simulink model "Coil"  (R2021b)
settings: Solver=FixedStepAuto  StartTime=-6000e-6  StopTime=6000e-6  FixedStep=25e-6  RelTol=1e-3
libraries: simulink x1
(part 1 of 2)
settings Model: Creator=teja  LastModifiedBy=teja

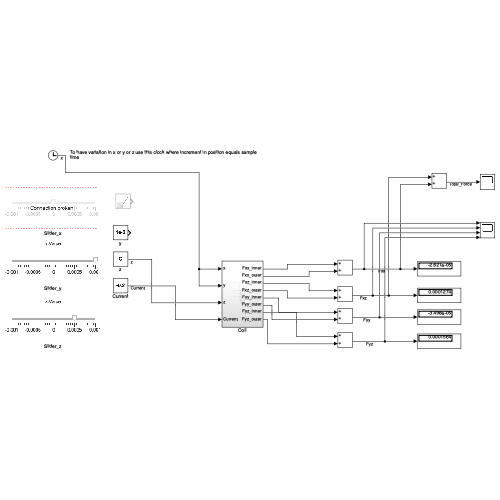
[thumbnail: Simulink's stored preview of the top-level diagram]
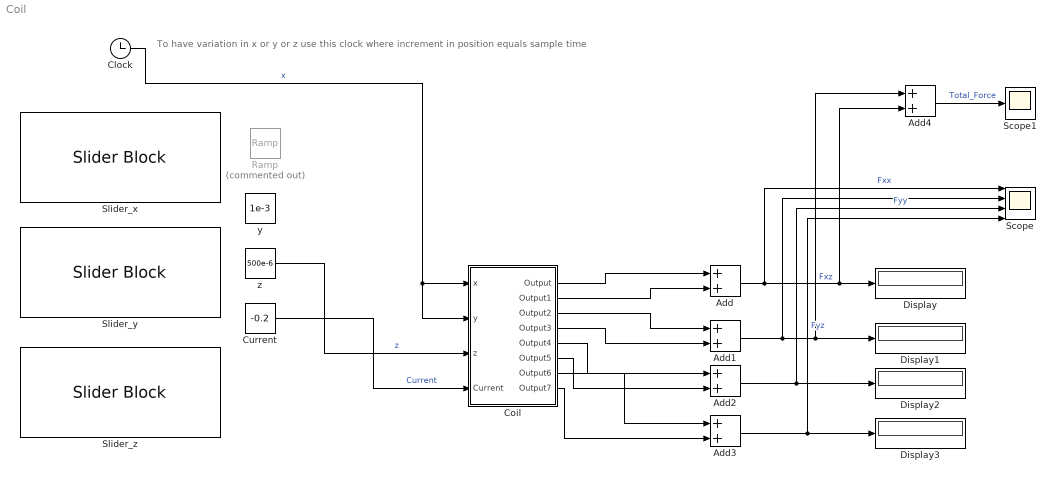
== system Coil ==
  note: To have variation in x or y or z use this clock where increment in position equals sample time
  Add{,1..4} (5 alike) : Sum
  Clock : Clock
  Coil : Subsystem
  Current : Constant  Value=-0.2
  Display{,1..3} (4 alike) : Display
  Ramp : simulink/Sources/Ramp  Commented=on  slope=1  start=0  InitialOutput=0
  Scope : Scope  NumInputPorts=4
  Scope1 : Scope
  Slider_x : SliderBlock  ScaleMin=-1000e-6  ScaleMax=1000e-6
  Slider_y : SliderBlock  ScaleMin=-1e-3  ScaleMax=1e-3
  Slider_z : SliderBlock  ScaleMin=-1000e-6  ScaleMax=1000e-6
  y : Constant  Value=1e-3
  z : Constant  Value=500e-6
  wires:
  Add/1 -> Add4/2, Display/1, Scope/1  "Fxx"
  Add1/1 -> Add4/1, Display1/1, Scope/2  "Fxz"
  Add2/1 -> Display2/1, Scope/3  "Fyy"
  Add3/1 -> Display3/1, Scope/4  "Fyz"
  Add4/1 -> Scope1/1  "Total_Force"
  z/1 -> Coil/3(z)  "z"
  Current/1 -> Coil/4(Current)  "Current"
  Coil/1(Output) -> Add/1
  Coil/2(Output1) -> Add/2
  Coil/3(Output2) -> Add1/1
  Coil/4(Output3) -> Add1/2
  Coil/5(Output4) -> Add2/1
  Coil/6(Output5) -> Add2/2
  Coil/7(Output6) -> Add3/1
  Coil/8(Output7) -> Add3/2
  Clock/1 -> Coil/1(x), Coil/2(y)  "x"

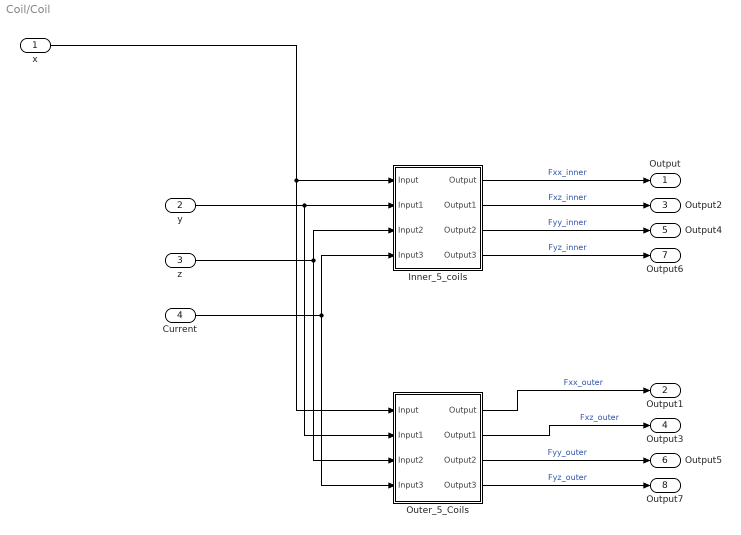
== system Coil/Coil ==
  x : Inport
  y : Inport  Port=2
  z : Inport  Port=3
  Current : Inport  Port=4
  Inner_5_coils : Subsystem
  Outer_5_Coils : Subsystem
  Output : Outport
  Output1 : Outport  Port=2
  Output2 : Outport  Port=3
  Output3 : Outport  Port=4
  Output4 : Outport  Port=5
  Output5 : Outport  Port=6
  Output6 : Outport  Port=7
  Output7 : Outport  Port=8
  wires:
  Outer_5_Coils/1(Output) -> Output1/1  "Fxx_outer"
  Inner_5_coils/4(Output3) -> Output6/1  "Fyz_inner"
  Outer_5_Coils/2(Output1) -> Output3/1  "Fxz_outer"
  y/1 -> Outer_5_Coils/2(Input1), Inner_5_coils/2(Input1)
  Outer_5_Coils/3(Output2) -> Output5/1  "Fyy_outer"
  z/1 -> Outer_5_Coils/3(Input2), Inner_5_coils/3(Input2)
  Inner_5_coils/2(Output1) -> Output2/1  "Fxz_inner"
  x/1 -> Outer_5_Coils/1(Input), Inner_5_coils/1(Input)
  Inner_5_coils/3(Output2) -> Output4/1  "Fyy_inner"
  Inner_5_coils/1(Output) -> Output/1  "Fxx_inner"
  Current/1 -> Outer_5_Coils/4(Input3), Inner_5_coils/4(Input3)
  Outer_5_Coils/4(Output3) -> Output7/1  "Fyz_outer"

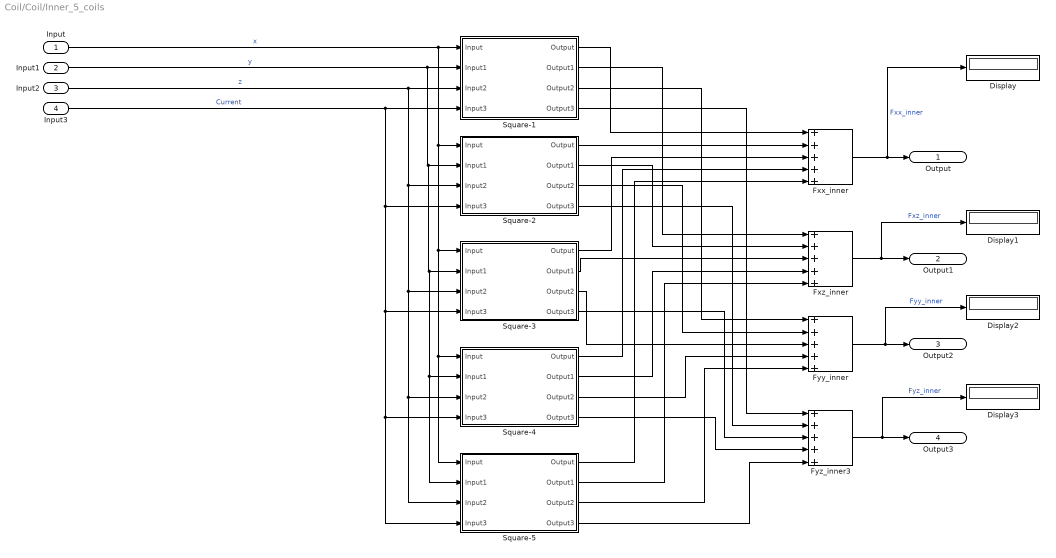
== system Coil/Coil/Inner_5_coils ==
  Input : Inport
  Input1 : Inport  Port=2
  Input2 : Inport  Port=3
  Input3 : Inport  Port=4
  Display{,1..3} (4 alike) : Display
  Fxx_inner : Sum  Inputs=+++++
  Fxz_inner : Sum  Inputs=+++++
  Fyy_inner : Sum  Inputs=+++++
  Fyz_inner3 : Sum  Inputs=+++++
  Square-1 : Subsystem
  Square-2 : Subsystem
  Square-3 : Subsystem
  Square-4 : Subsystem
  Square-5 : Subsystem
  Output : Outport
  Output1 : Outport  Port=2
  Output2 : Outport  Port=3
  Output3 : Outport  Port=4
  wires:
  Input/1 -> Square-5/1(Input), Square-4/1(Input), Square-3/1(Input), Square-2/1(Input), Square-1/1(Input)  "x"
  Input3/1 -> Square-2/4(Input3), Square-3/4(Input3), Square-4/4(Input3), Square-5/4(Input3), Square-1/4(Input3)  "Current"
  Input1/1 -> Square-5/2(Input1), Square-4/2(Input1), Square-3/2(Input1), Square-2/2(Input1), Square-1/2(Input1)  "y"
  Input2/1 -> Square-1/3(Input2), Square-3/3(Input2), Square-4/3(Input2), Square-5/3(Input2), Square-2/3(Input2)  "z"
  Square-1/1(Output) -> Fxx_inner/1
  Square-2/1(Output) -> Fxx_inner/2
  Square-3/1(Output) -> Fxx_inner/3
  Square-4/1(Output) -> Fxx_inner/4
  Square-5/1(Output) -> Fxx_inner/5
  Fxx_inner/1 -> Display/1, Output/1  "Fxx_inner"
  Fxz_inner/1 -> Display1/1, Output1/1  "Fxz_inner"
  Fyy_inner/1 -> Display2/1, Output2/1  "Fyy_inner"
  Fyz_inner3/1 -> Display3/1, Output3/1  "Fyz_inner"
  Square-1/2(Output1) -> Fxz_inner/1
  Square-2/2(Output1) -> Fxz_inner/2
  Square-3/2(Output1) -> Fxz_inner/3
  Square-4/2(Output1) -> Fxz_inner/4
  Square-5/2(Output1) -> Fxz_inner/5
  Square-1/3(Output2) -> Fyy_inner/1
  Square-2/3(Output2) -> Fyy_inner/2
  Square-3/3(Output2) -> Fyy_inner/3
  Square-4/3(Output2) -> Fyy_inner/4
  Square-5/3(Output2) -> Fyy_inner/5
  Square-1/4(Output3) -> Fyz_inner3/1
  Square-2/4(Output3) -> Fyz_inner3/2
  Square-3/4(Output3) -> Fyz_inner3/3
  Square-4/4(Output3) -> Fyz_inner3/4
  Square-5/4(Output3) -> Fyz_inner3/5

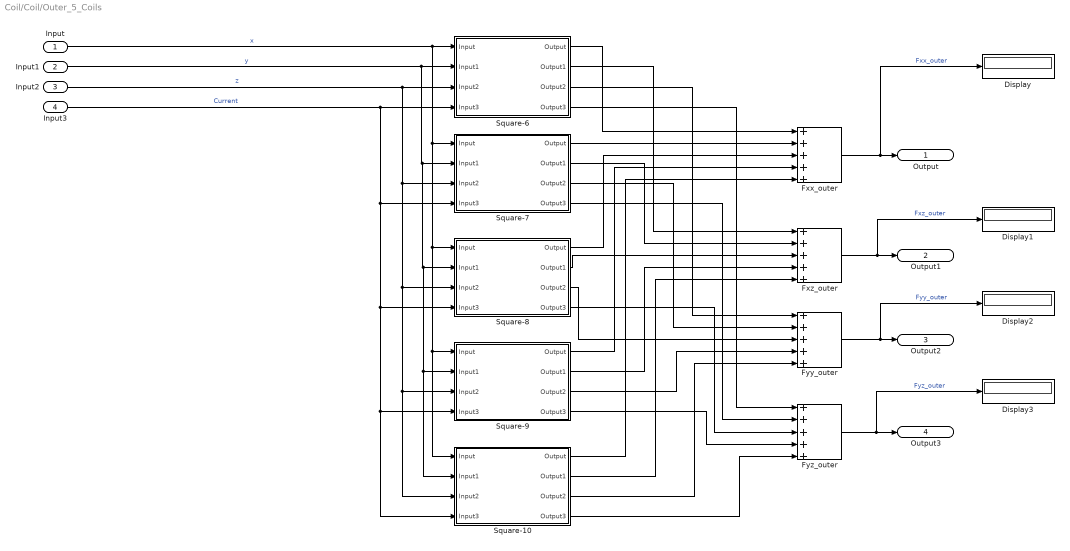
== system Coil/Coil/Outer_5_Coils ==
  Input : Inport
  Input1 : Inport  Port=2
  Input2 : Inport  Port=3
  Input3 : Inport  Port=4
  Display{,1..3} (4 alike) : Display
  Fxx_outer : Sum  Inputs=+++++
  Fxz_outer : Sum  Inputs=+++++
  Fyy_outer : Sum  Inputs=+++++
  Fyz_outer : Sum  Inputs=+++++
  Square-10 : Subsystem
  Square-6 : Subsystem
  Square-7 : Subsystem
  Square-8 : Subsystem
  Square-9 : Subsystem
  Output : Outport
  Output1 : Outport  Port=2
  Output2 : Outport  Port=3
  Output3 : Outport  Port=4
  wires:
  Square-10/4(Output3) -> Fyz_outer/5
  Square-9/4(Output3) -> Fyz_outer/4
  Square-8/4(Output3) -> Fyz_outer/3
  Square-7/4(Output3) -> Fyz_outer/2
  Square-6/4(Output3) -> Fyz_outer/1
  Square-10/3(Output2) -> Fyy_outer/5
  Square-9/3(Output2) -> Fyy_outer/4
  Square-8/3(Output2) -> Fyy_outer/3
  Square-7/3(Output2) -> Fyy_outer/2
  Square-6/3(Output2) -> Fyy_outer/1
  Square-10/2(Output1) -> Fxz_outer/5
  Square-9/2(Output1) -> Fxz_outer/4
  Square-8/2(Output1) -> Fxz_outer/3
  Square-7/2(Output1) -> Fxz_outer/2
  Square-6/2(Output1) -> Fxz_outer/1
  Fyz_outer/1 -> Display3/1, Output3/1  "Fyz_outer"
  Fyy_outer/1 -> Display2/1, Output2/1  "Fyy_outer"
  Fxz_outer/1 -> Display1/1, Output1/1  "Fxz_outer"
  Fxx_outer/1 -> Display/1, Output/1  "Fxx_outer"
  Square-10/1(Output) -> Fxx_outer/5
  Square-9/1(Output) -> Fxx_outer/4
  Square-8/1(Output) -> Fxx_outer/3
  Square-7/1(Output) -> Fxx_outer/2
  Square-6/1(Output) -> Fxx_outer/1
  Input2/1 -> Square-7/3(Input2), Square-10/3(Input2), Square-9/3(Input2), Square-8/3(Input2), Square-6/3(Input2)  "z"
  Input1/1 -> Square-6/2(Input1), Square-7/2(Input1), Square-8/2(Input1), Square-9/2(Input1), Square-10/2(Input1)  "y"
  Input3/1 -> Square-6/4(Input3), Square-10/4(Input3), Square-9/4(Input3), Square-8/4(Input3), Square-7/4(Input3)  "Current"
  Input/1 -> Square-6/1(Input), Square-7/1(Input), Square-8/1(Input), Square-9/1(Input), Square-10/1(Input)  "x"

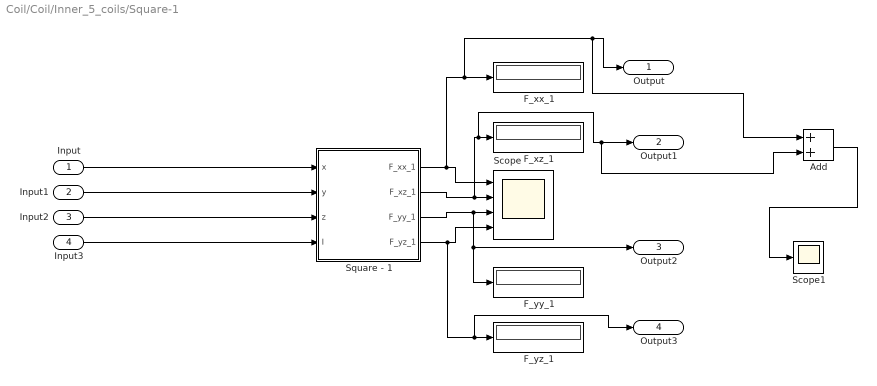
== system Coil/Coil/Inner_5_coils/Square-1 ==
  Input : Inport
  Input1 : Inport  Port=2
  Input2 : Inport  Port=3
  Input3 : Inport  Port=4
  Add : Sum
  F_xx_1 : Display
  F_xz_1 : Display
  F_yy_1 : Display
  F_yz_1 : Display
  Scope : Scope  NumInputPorts=4
  Scope1 : Scope
  Square - 1 : MATLAB Function  TreatAsAtomicUnit=on
  Output : Outport
  Output1 : Outport  Port=2
  Output2 : Outport  Port=3
  Output3 : Outport  Port=4
  wires:
  Square - 1/2(F_xz_1) -> Add/2, Output1/1, F_xz_1/1, Scope/2
  Square - 1/3(F_yy_1) -> F_yy_1/1, Output2/1, Scope/3
  Square - 1/1(F_xx_1) -> Add/1, Output/1, F_xx_1/1, Scope/1
  Square - 1/4(F_yz_1) -> Scope/4, Output3/1, F_yz_1/1
  Input/1 -> Square - 1/1(x)
  Input1/1 -> Square - 1/2(y)
  Input2/1 -> Square - 1/3(z)
  Input3/1 -> Square - 1/4(I)
  Add/1 -> Scope1/1

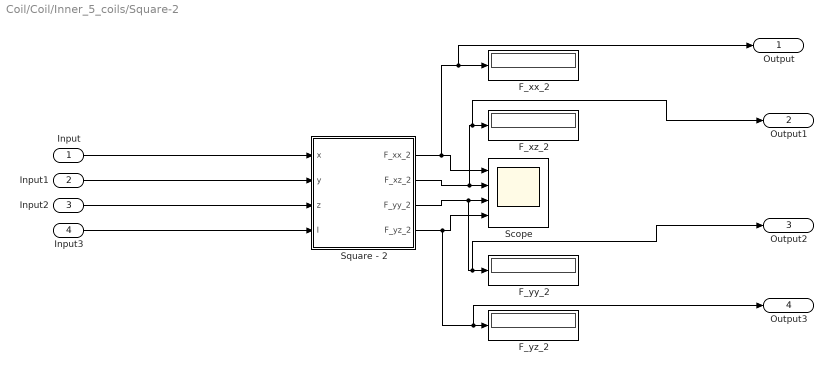
== system Coil/Coil/Inner_5_coils/Square-2 ==
  Input : Inport
  Input1 : Inport  Port=2
  Input2 : Inport  Port=3
  Input3 : Inport  Port=4
  F_xx_2 : Display
  F_xz_2 : Display
  F_yy_2 : Display
  F_yz_2 : Display
  Scope : Scope  NumInputPorts=4
  Square - 2 : MATLAB Function  TreatAsAtomicUnit=on
  Output : Outport
  Output1 : Outport  Port=2
  Output2 : Outport  Port=3
  Output3 : Outport  Port=4
  wires:
  Square - 2/1(F_xx_2) -> Scope/1, Output/1, F_xx_2/1
  Square - 2/2(F_xz_2) -> Scope/2, Output1/1, F_xz_2/1
  Square - 2/4(F_yz_2) -> Scope/4, Output3/1, F_yz_2/1
  Square - 2/3(F_yy_2) -> Scope/3, Output2/1, F_yy_2/1
  Input2/1 -> Square - 2/3(z)
  Input1/1 -> Square - 2/2(y)
  Input/1 -> Square - 2/1(x)
  Input3/1 -> Square - 2/4(I)

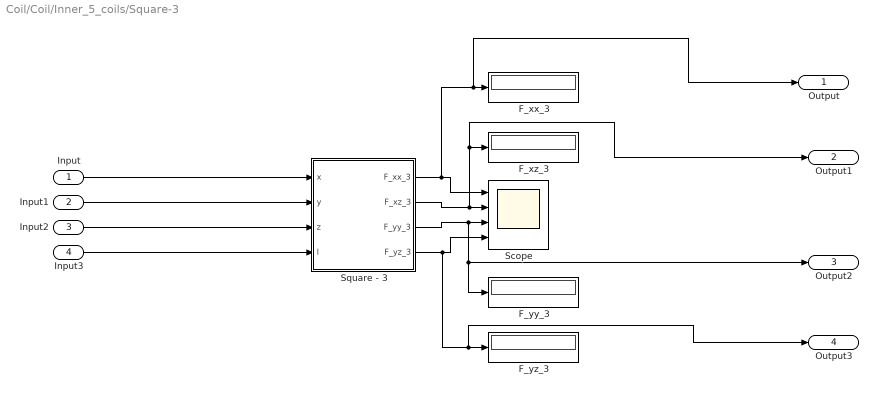
== system Coil/Coil/Inner_5_coils/Square-3 ==
  Input : Inport
  Input1 : Inport  Port=2
  Input2 : Inport  Port=3
  Input3 : Inport  Port=4
  F_xx_3 : Display
  F_xz_3 : Display
  F_yy_3 : Display
  F_yz_3 : Display
  Scope : Scope  NumInputPorts=4
  Square - 3 : MATLAB Function  TreatAsAtomicUnit=on
  Output : Outport
  Output1 : Outport  Port=2
  Output2 : Outport  Port=3
  Output3 : Outport  Port=4
  wires:
  Square - 3/1(F_xx_3) -> Scope/1, Output/1, F_xx_3/1
  Square - 3/4(F_yz_3) -> Scope/4, Output3/1, F_yz_3/1
  Square - 3/2(F_xz_3) -> Scope/2, Output1/1, F_xz_3/1
  Square - 3/3(F_yy_3) -> Scope/3, F_yy_3/1, Output2/1
  Input2/1 -> Square - 3/3(z)
  Input1/1 -> Square - 3/2(y)
  Input/1 -> Square - 3/1(x)
  Input3/1 -> Square - 3/4(I)

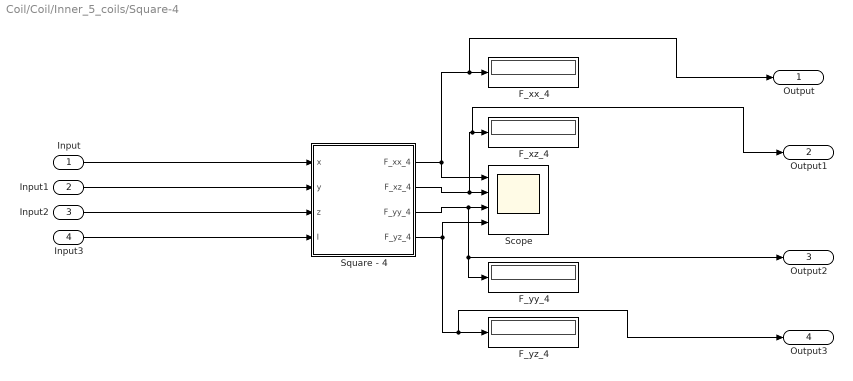
== system Coil/Coil/Inner_5_coils/Square-4 ==
  Input : Inport
  Input1 : Inport  Port=2
  Input2 : Inport  Port=3
  Input3 : Inport  Port=4
  F_xx_4 : Display
  F_xz_4 : Display
  F_yy_4 : Display
  F_yz_4 : Display
  Scope : Scope  NumInputPorts=4
  Square - 4 : MATLAB Function  TreatAsAtomicUnit=on
  Output : Outport
  Output1 : Outport  Port=2
  Output2 : Outport  Port=3
  Output3 : Outport  Port=4
  wires:
  Square - 4/1(F_xx_4) -> Scope/1, Output/1, F_xx_4/1
  Square - 4/4(F_yz_4) -> Scope/4, Output3/1, F_yz_4/1
  Square - 4/2(F_xz_4) -> Output1/1, F_xz_4/1, Scope/2
  Square - 4/3(F_yy_4) -> Scope/3, Output2/1, F_yy_4/1
  Input2/1 -> Square - 4/3(z)
  Input1/1 -> Square - 4/2(y)
  Input/1 -> Square - 4/1(x)
  Input3/1 -> Square - 4/4(I)

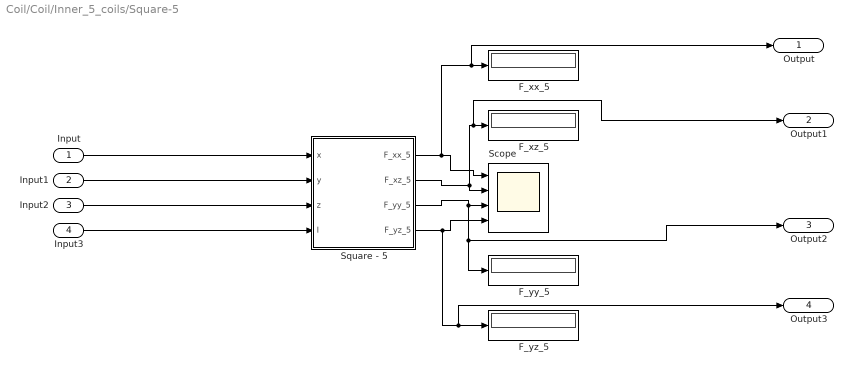
== system Coil/Coil/Inner_5_coils/Square-5 ==
  Input : Inport
  Input1 : Inport  Port=2
  Input2 : Inport  Port=3
  Input3 : Inport  Port=4
  F_xx_5 : Display
  F_xz_5 : Display
  F_yy_5 : Display
  F_yz_5 : Display
  Scope : Scope  NumInputPorts=4
  Square - 5 : MATLAB Function  TreatAsAtomicUnit=on
  Output : Outport
  Output1 : Outport  Port=2
  Output2 : Outport  Port=3
  Output3 : Outport  Port=4
  wires:
  Square - 5/1(F_xx_5) -> Scope/1, Output/1, F_xx_5/1
  Square - 5/4(F_yz_5) -> Scope/4, Output3/1, F_yz_5/1
  Square - 5/2(F_xz_5) -> Scope/2, Output1/1, F_xz_5/1
  Square - 5/3(F_yy_5) -> Scope/3, Output2/1, F_yy_5/1
  Input2/1 -> Square - 5/3(z)
  Input1/1 -> Square - 5/2(y)
  Input/1 -> Square - 5/1(x)
  Input3/1 -> Square - 5/4(I)

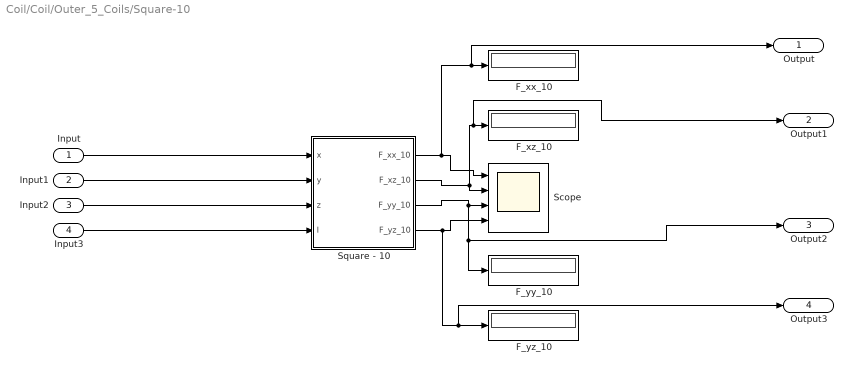
== system Coil/Coil/Outer_5_Coils/Square-10 ==
  Input : Inport
  Input1 : Inport  Port=2
  Input2 : Inport  Port=3
  Input3 : Inport  Port=4
  F_xx_10 : Display
  F_xz_10 : Display
  F_yy_10 : Display
  F_yz_10 : Display
  Scope : Scope  NumInputPorts=4
  Square - 10 : MATLAB Function  TreatAsAtomicUnit=on
  Output : Outport
  Output1 : Outport  Port=2
  Output2 : Outport  Port=3
  Output3 : Outport  Port=4
  wires:
  Input3/1 -> Square - 10/4(I)
  Input/1 -> Square - 10/1(x)
  Input1/1 -> Square - 10/2(y)
  Input2/1 -> Square - 10/3(z)
  Square - 10/3(F_yy_10) -> Scope/3, F_yy_10/1, Output2/1
  Square - 10/2(F_xz_10) -> Scope/2, F_xz_10/1, Output1/1
  Square - 10/4(F_yz_10) -> Scope/4, F_yz_10/1, Output3/1
  Square - 10/1(F_xx_10) -> Scope/1, F_xx_10/1, Output/1

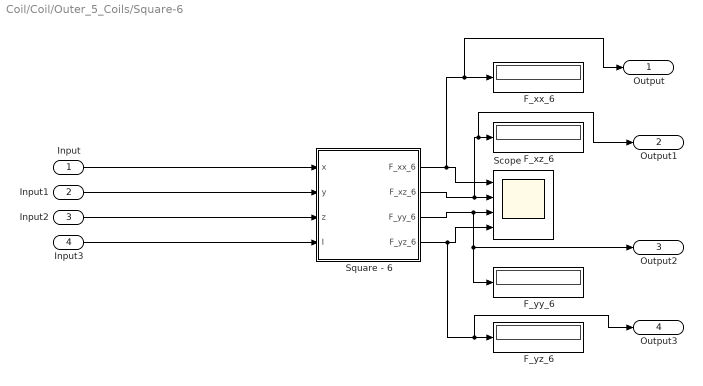
== system Coil/Coil/Outer_5_Coils/Square-6 ==
  Input : Inport
  Input1 : Inport  Port=2
  Input2 : Inport  Port=3
  Input3 : Inport  Port=4
  F_xx_6 : Display
  F_xz_6 : Display
  F_yy_6 : Display
  F_yz_6 : Display
  Scope : Scope  NumInputPorts=4
  Square - 6 : MATLAB Function  TreatAsAtomicUnit=on
  Output : Outport
  Output1 : Outport  Port=2
  Output2 : Outport  Port=3
  Output3 : Outport  Port=4
  wires:
  Input3/1 -> Square - 6/4(I)
  Input2/1 -> Square - 6/3(z)
  Input1/1 -> Square - 6/2(y)
  Input/1 -> Square - 6/1(x)
  Square - 6/4(F_yz_6) -> Scope/4, F_yz_6/1, Output3/1
  Square - 6/1(F_xx_6) -> Scope/1, F_xx_6/1, Output/1
  Square - 6/3(F_yy_6) -> Scope/3, Output2/1, F_yy_6/1
  Square - 6/2(F_xz_6) -> Scope/2, F_xz_6/1, Output1/1

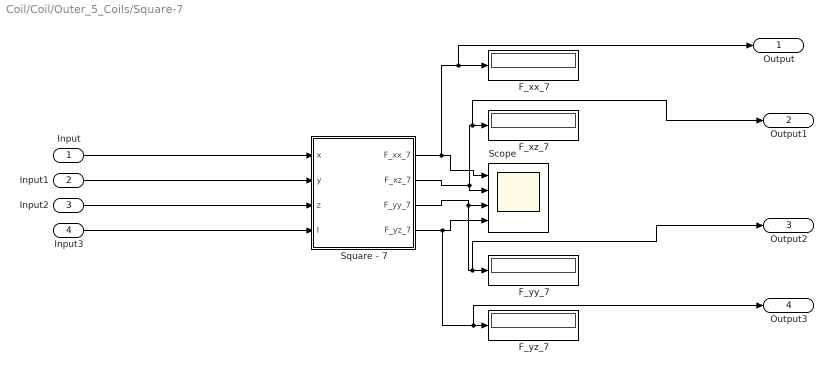
== system Coil/Coil/Outer_5_Coils/Square-7 ==
  Input : Inport
  Input1 : Inport  Port=2
  Input2 : Inport  Port=3
  Input3 : Inport  Port=4
  F_xx_7 : Display
  F_xz_7 : Display
  F_yy_7 : Display
  F_yz_7 : Display
  Scope : Scope  NumInputPorts=4
  Square - 7 : MATLAB Function  TreatAsAtomicUnit=on
  Output : Outport
  Output1 : Outport  Port=2
  Output2 : Outport  Port=3
  Output3 : Outport  Port=4
  wires:
  Input3/1 -> Square - 7/4(I)
  Input/1 -> Square - 7/1(x)
  Input1/1 -> Square - 7/2(y)
  Input2/1 -> Square - 7/3(z)
  Square - 7/3(F_yy_7) -> Scope/3, F_yy_7/1, Output2/1
  Square - 7/4(F_yz_7) -> Scope/4, F_yz_7/1, Output3/1
  Square - 7/2(F_xz_7) -> Scope/2, F_xz_7/1, Output1/1
  Square - 7/1(F_xx_7) -> Scope/1, F_xx_7/1, Output/1

== system Coil/Coil/Outer_5_Coils/Square-8 ==
  Input : Inport
  Input1 : Inport  Port=2
  Input2 : Inport  Port=3
  Input3 : Inport  Port=4
  F_xx_8 : Display
  F_xz_8 : Display
  F_yy_8 : Display
  F_yz_8 : Display
  Scope : Scope  NumInputPorts=4
  Square - 8 : MATLAB Function  TreatAsAtomicUnit=on
  Output : Outport
  Output1 : Outport  Port=2
  Output2 : Outport  Port=3
  Output3 : Outport  Port=4
  wires:
  Input3/1 -> Square - 8/4(I)
  Input/1 -> Square - 8/1(x)
  Input1/1 -> Square - 8/2(y)
  Input2/1 -> Square - 8/3(z)
  Square - 8/3(F_yy_8) -> Scope/3, Output2/1, F_yy_8/1
  Square - 8/2(F_xz_8) -> Scope/2, F_xz_8/1, Output1/1
  Square - 8/4(F_yz_8) -> Scope/4, F_yz_8/1, Output3/1
  Square - 8/1(F_xx_8) -> Scope/1, F_xx_8/1, Output/1

== system Coil/Coil/Outer_5_Coils/Square-9 ==
  Input : Inport
  Input1 : Inport  Port=2
  Input2 : Inport  Port=3
  Input3 : Inport  Port=4
  F_xx_9 : Display
  F_xz_9 : Display
  F_yy_9 : Display
  F_yz_9 : Display
  Scope : Scope  NumInputPorts=4
  Square - 9 : MATLAB Function  TreatAsAtomicUnit=on
  Output : Outport
  Output1 : Outport  Port=2
  Output2 : Outport  Port=3
  Output3 : Outport  Port=4
  wires:
  Input3/1 -> Square - 9/4(I)
  Input/1 -> Square - 9/1(x)
  Input1/1 -> Square - 9/2(y)
  Input2/1 -> Square - 9/3(z)
  Square - 9/3(F_yy_9) -> Scope/3, F_yy_9/1, Output2/1
  Square - 9/2(F_xz_9) -> Scope/2, F_xz_9/1, Output1/1
  Square - 9/4(F_yz_9) -> Scope/4, F_yz_9/1, Output3/1
  Square - 9/1(F_xx_9) -> Scope/1, F_xx_9/1, Output/1

== matlab function Coil/Outer_5_Coils/Square-8/Square - 8 ==
  data: x input; F_xx_8 output; F_xz_8 output; y input; z input; I input; F_yy_8 output; F_yz_8 output
function [F_xx_8, F_xz_8, F_yy_8, F_yz_8] = force(x, y, z, I)

g = 415e-6;     %Coil spacing
m0 = 4*pi*1e-7;
radius = 3e-3;%m
height = 1e-3;%m
Magentization = 1.45; %T
vol_cy = pi*radius^2*height; %If Object is Cylinder, vol in m^3
% vol_sp = (4/3)*(pi * radius^3); %If Object is Sphere, vol in m^3

k = 0.4e-3; %additional length added to wires, to get concentric coil
%--------%--------%--------%--------%--------%--------%--------%----------
% Line along y - axis
%-%--------%--------%--------%--------%--------%--------%--------%--------
yp1_1 = -0.6e-3 - 7*k;
yp2_1 = 0.6e-3 + 7*k;
yn1_1 = -0.8e-3 - 7*k;
yn2_1 = 0.8e-3 + 7*k;
a_xp_1 = 8*g;  
a_xn_1 = -8*g;

k_yp_1 = 1/(4*pi*((a_xp_1-x)^2+z^2));
k_1yp_1 = (yp2_1-y)/((yp2_1-y)^2+(a_xp_1-x)^2+z^2)^0.5;
k_2yp_1 = (yp1_1-y)/((yp1_1-y)^2+(a_xp_1-x)^2+z^2)^0.5;

k_1yp_3 = (yp2_1-y)/((yp2_1-y)^2+(a_xp_1-x)^2+z^2)^1.5;
k_2yp_3 = (yp1_1-y)/((yp1_1-y)^2+(a_xp_1-x)^2+z^2)^1.5;

k_yn_1 = 1/(4*pi*((a_xn_1-x)^2+z^2));
k_1yn_1 = (yn2_1-y)/((yn2_1-y)^2+(a_xn_1-x)^2+z^2)^0.5;
k_2yn_1 = (yn1_1-y)/((yn1_1-y)^2+(a_xn_1-x)^2+z^2)^0.5;

k_1yn_3 = (yn2_1-y)/((yn2_1-y)^2+(a_xn_1-x)^2+z^2)^1.5;
k_2yn_3 = (yn1_1-y)/((yn1_1-y)^2+(a_xn_1-x)^2+z^2)^1.5;

hyp_x_1 = -(z*k_yp_1*(a_xp_1-x))*I*m0;
hyp_x1_1 = (k_yp_1*(k_1yp_1 - k_2yp_1))*2*4*pi;
hyp_x2_1 = k_1yp_3 - k_2yp_3;
dBxp_1_dx = hyp_x_1*(hyp_x1_1 + hyp_x2_1);

hyp_z_1 = (k_yp_1)*I*m0;
hyp_z1_1 = (k_1yp_1 - k_2yp_1)*(-1);
hyp_z2_1 = (k_yp_1*(k_1yp_1 - k_2yp_1)*(z^2))*4*pi*2;
hyp_z3_1 = (k_1yp_3 - k_2yp_3)*(z^2);
dBxp_1_dz = hyp_z_1*(hyp_z1_1 + hyp_z2_1 + hyp_z3_1);

hyn_x_1 = -(z*k_yn_1*(a_xn_1-x))*I*m0*(-1);
hyn_x1_1 = (k_yn_1*(k_1yn_1 - k_2yn_1))*2*4*pi;
hyn_x2_1 = k_1yn_3 - k_2yn_3;
dBxn_1_dx = hyn_x_1*(hyn_x1_1 + hyn_x2_1);

hyn_z_1 = (k_yn_1)*I*m0*(-1);
hyn_z1_1 = (k_1yn_1 - k_2yn_1)*(-1);
hyn_z2_1 = (k_yn_1*(k_1yn_1 - k_2yn_1)*(z^2))*4*pi*2;
hyn_z3_1 = (k_1yn_3 - k_2yn_3)*(z^2);
dBxn_1_dz = hyn_z_1*(hyn_z1_1 + hyn_z2_1 + hyn_z3_1);

%--------%--------%--------%--------%--------%--------%--------%----------
% Line along x - axis
%-%--------%--------%--------%--------%a--------%--------%--------%--------
xp1_1 = -0.8e-3 - 7*k;
xp2_1 = 0.8e-3 + 7*k;
xn1_1 = -1e-3 - 7*k;
xn2_1 = 1e-3 + 7*k;
a_yp_1 = 3.475e-3;          %Distance of coil from (0,0)
a_yn_1 = -3.475e-3;

k_xp_1 = 1/(4*pi*((a_yp_1-y)^2+z^2));
k_1xp_1 = (xp2_1-x)/((xp2_1-x)^2+(a_yp_1-y)^2+z^2)^0.5;
k_2xp_1 = (xp1_1-x)/((xp1_1-x)^2+(a_yp_1-y)^2+z^2)^0.5;

k_xn_1 = 1/(4*pi*((a_yn_1-y)^2+z^2));
k_1xn_1 = (xn2_1-x)/((xn2_1-x)^2+(a_yn_1-y)^2+z^2)^0.5;
k_2xn_1 = (xn1_1-x)/((xn1_1-x)^2+(a_yn_1-y)^2+z^2)^0.5;

k_1xp_3 = (xp2_1-x)/((xp2_1-x)^2+(a_yp_1-y)^2+z^2)^1.5;
k_2xp_3 = (xp1_1-x)/((xp1_1-x)^2+(a_yp_1-y)^2+z^2)^1.5;

k_1xn_3 = (xn2_1-x)/((xn2_1-x)^2+(a_yn_1-y)^2+z^2)^1.5;
k_2xn_3 = (xn1_1-x)/((xn1_1-x)^2+(a_yn_1-y)^2+z^2)^1.5;

hxp_x_1 = -(z*k_xp_1*(a_yp_1-y))*I*m0;
hxp_x1_1 = (k_xp_1*(k_1xp_1 - k_2xp_1))*2*4*pi;
hxp_x2_1 = k_1xp_3 - k_2xp_3;
dByp_1_dy = hxp_x_1*(hxp_x1_1 + hxp_x2_1);

hxp_z_1 = (k_xp_1)*I*m0;
hxp_z1_1 = (k_1xp_1 - k_2xp_1)*(-1);
hxp_z2_1 = (k_xp_1*(k_1xp_1 - k_2xp_1)*(z^2))*4*pi*2;
hxp_z3_1 = (k_1xp_3 - k_2xp_3)*(z^2);
dByp_1_dz = hxp_z_1*(hxp_z1_1 + hxp_z2_1 + hxp_z3_1);

hxn_x_1 = -(z*k_xn_1*(a_yn_1-y))*I*m0*(-1);
hxn_x1_1 = (k_xn_1*(k_1xn_1 - k_2xn_1))*2*4*pi;
hxn_x2_1 = k_1xn_3 - k_2xn_3;
dByn_1_dy = hxn_x_1*(hxn_x1_1 + hxn_x2_1);

hxn_z_1 = (k_xn_1)*I*m0*(-1);
hxn_z1_1 = (k_1xn_1 - k_2xn_1)*(-1);
hxn_z2_1 = (k_xn_1*(k_1xn_1 - k_2xn_1)*(z^2))*4*pi*2;
hxn_z3_1 = (k_1xn_3 - k_2xn_3)*(z^2);
dByn_1_dz = hxn_z_1*(hxn_z1_1 + hxn_z2_1 + hxn_z3_1);

F_xx_8 = vol_cy * Magentization* (dBxp_1_dx + dBxn_1_dx)/m0;
F_xz_8 = vol_cy * Magentization* (dBxp_1_dz + dBxn_1_dz)/m0;
F_yy_8 = vol_cy * Magentization* (dByp_1_dy + dByn_1_dy)/m0;
F_yz_8 = vol_cy * Magentization* (dByp_1_dz + dByn_1_dz)/m0;
end

== matlab function Coil/Outer_5_Coils/Square-9/Square - 9 ==
  data: x input; F_xx_9 output; F_xz_9 output; y input; z input; I input; F_yy_9 output; F_yz_9 output
function [F_xx_9, F_xz_9, F_yy_9, F_yz_9] = force(x, y, z, I)

g = 413.33e-6;     %Coil spacing
m0 = 4*pi*1e-7;
radius = 3e-3;%m
height = 1e-3;%m
Magentization = 1.45; %T
vol_cy = pi*radius^2*height; %If Object is Cylinder, vol in m^3
% vol_sp = (4/3)*(pi * radius^3); %If Object is Sphere, vol in m^3

k = 0.4e-3; %additional length added to wires, to get concentric coil
%--------%--------%--------%--------%--------%--------%--------%----------
% Line along y - axis
%-%--------%--------%--------%--------%--------%--------%--------%--------
yp1_1 = -0.6e-3 - 8*k;
yp2_1 = 0.6e-3 + 8*k;
yn1_1 = -0.8e-3 - 8*k;
yn2_1 = 0.8e-3 + 8*k;
a_xp_1 = 9*g;  
a_xn_1 = -9*g;

k_yp_1 = 1/(4*pi*((a_xp_1-x)^2+z^2));
k_1yp_1 = (yp2_1-y)/((yp2_1-y)^2+(a_xp_1-x)^2+z^2)^0.5;
k_2yp_1 = (yp1_1-y)/((yp1_1-y)^2+(a_xp_1-x)^2+z^2)^0.5;

k_1yp_3 = (yp2_1-y)/((yp2_1-y)^2+(a_xp_1-x)^2+z^2)^1.5;
k_2yp_3 = (yp1_1-y)/((yp1_1-y)^2+(a_xp_1-x)^2+z^2)^1.5;

k_yn_1 = 1/(4*pi*((a_xn_1-x)^2+z^2));
k_1yn_1 = (yn2_1-y)/((yn2_1-y)^2+(a_xn_1-x)^2+z^2)^0.5;
k_2yn_1 = (yn1_1-y)/((yn1_1-y)^2+(a_xn_1-x)^2+z^2)^0.5;

k_1yn_3 = (yn2_1-y)/((yn2_1-y)^2+(a_xn_1-x)^2+z^2)^1.5;
k_2yn_3 = (yn1_1-y)/((yn1_1-y)^2+(a_xn_1-x)^2+z^2)^1.5;

hyp_x_1 = -(z*k_yp_1*(a_xp_1-x))*I*m0;
hyp_x1_1 = (k_yp_1*(k_1yp_1 - k_2yp_1))*2*4*pi;
hyp_x2_1 = k_1yp_3 - k_2yp_3;
dBxp_1_dx = hyp_x_1*(hyp_x1_1 + hyp_x2_1);

hyp_z_1 = (k_yp_1)*I*m0;
hyp_z1_1 = (k_1yp_1 - k_2yp_1)*(-1);
hyp_z2_1 = (k_yp_1*(k_1yp_1 - k_2yp_1)*(z^2))*4*pi*2;
hyp_z3_1 = (k_1yp_3 - k_2yp_3)*(z^2);
dBxp_1_dz = hyp_z_1*(hyp_z1_1 + hyp_z2_1 + hyp_z3_1);

hyn_x_1 = -(z*k_yn_1*(a_xn_1-x))*I*m0*(-1);
hyn_x1_1 = (k_yn_1*(k_1yn_1 - k_2yn_1))*2*4*pi;
hyn_x2_1 = k_1yn_3 - k_2yn_3;
dBxn_1_dx = hyn_x_1*(hyn_x1_1 + hyn_x2_1);

hyn_z_1 = (k_yn_1)*I*m0*(-1);
hyn_z1_1 = (k_1yn_1 - k_2yn_1)*(-1);
hyn_z2_1 = (k_yn_1*(k_1yn_1 - k_2yn_1)*(z^2))*4*pi*2;
hyn_z3_1 = (k_1yn_3 - k_2yn_3)*(z^2);
dBxn_1_dz = hyn_z_1*(hyn_z1_1 + hyn_z2_1 + hyn_z3_1);

%--------%--------%--------%--------%--------%--------%--------%----------
% Line along x - axis
%-%--------%--------%--------%--------%a--------%--------%--------%--------
xp1_1 = -0.8e-3 - 8*k;
xp2_1 = 0.8e-3 + 8*k;
xn1_1 = -1e-3 - 8*k;
xn2_1 = 1e-3 + 8*k;
a_yp_1 = 3.875e-3;          %Distance of coil from (0,0)
a_yn_1 = -3.875e-3;

k_xp_1 = 1/(4*pi*((a_yp_1-y)^2+z^2));
k_1xp_1 = (xp2_1-x)/((xp2_1-x)^2+(a_yp_1-y)^2+z^2)^0.5;
k_2xp_1 = (xp1_1-x)/((xp1_1-x)^2+(a_yp_1-y)^2+z^2)^0.5;

k_xn_1 = 1/(4*pi*((a_yn_1-y)^2+z^2));
k_1xn_1 = (xn2_1-x)/((xn2_1-x)^2+(a_yn_1-y)^2+z^2)^0.5;
k_2xn_1 = (xn1_1-x)/((xn1_1-x)^2+(a_yn_1-y)^2+z^2)^0.5;

k_1xp_3 = (xp2_1-x)/((xp2_1-x)^2+(a_yp_1-y)^2+z^2)^1.5;
k_2xp_3 = (xp1_1-x)/((xp1_1-x)^2+(a_yp_1-y)^2+z^2)^1.5;

k_1xn_3 = (xn2_1-x)/((xn2_1-x)^2+(a_yn_1-y)^2+z^2)^1.5;
k_2xn_3 = (xn1_1-x)/((xn1_1-x)^2+(a_yn_1-y)^2+z^2)^1.5;

hxp_x_1 = -(z*k_xp_1*(a_yp_1-y))*I*m0;
hxp_x1_1 = (k_xp_1*(k_1xp_1 - k_2xp_1))*2*4*pi;
hxp_x2_1 = k_1xp_3 - k_2xp_3;
dByp_1_dy = hxp_x_1*(hxp_x1_1 + hxp_x2_1);

hxp_z_1 = (k_xp_1)*I*m0;
hxp_z1_1 = (k_1xp_1 - k_2xp_1)*(-1);
hxp_z2_1 = (k_xp_1*(k_1xp_1 - k_2xp_1)*(z^2))*4*pi*2;
hxp_z3_1 = (k_1xp_3 - k_2xp_3)*(z^2);
dByp_1_dz = hxp_z_1*(hxp_z1_1 + hxp_z2_1 + hxp_z3_1);

hxn_x_1 = -(z*k_xn_1*(a_yn_1-y))*I*m0*(-1);
hxn_x1_1 = (k_xn_1*(k_1xn_1 - k_2xn_1))*2*4*pi;
hxn_x2_1 = k_1xn_3 - k_2xn_3;
dByn_1_dy = hxn_x_1*(hxn_x1_1 + hxn_x2_1);

hxn_z_1 = (k_xn_1)*I*m0*(-1);
hxn_z1_1 = (k_1xn_1 - k_2xn_1)*(-1);
hxn_z2_1 = (k_xn_1*(k_1xn_1 - k_2xn_1)*(z^2))*4*pi*2;
hxn_z3_1 = (k_1xn_3 - k_2xn_3)*(z^2);
dByn_1_dz = hxn_z_1*(hxn_z1_1 + hxn_z2_1 + hxn_z3_1);

F_xx_9 = vol_cy * Magentization* (dBxp_1_dx + dBxn_1_dx)/m0;
F_xz_9 = vol_cy * Magentization* (dBxp_1_dz + dBxn_1_dz)/m0;
F_yy_9 = vol_cy * Magentization* (dByp_1_dy + dByn_1_dy)/m0;
F_yz_9 = vol_cy * Magentization* (dByp_1_dz + dByn_1_dz)/m0;
end

== matlab function Coil/Inner_5_coils/Square-2/Square - 2 ==
  data: x input; F_xx_2 output; F_xz_2 output; y input; z input; I input; F_yy_2 output; F_yz_2 output
function [F_xx_2, F_xz_2, F_yy_2, F_yz_2] = force(x, y, z, I)

g = 460e-6;     %Coil spacing
m0 = 4*pi*1e-7;
radius = 3e-3;%m
height = 1e-3;%m
Magentization = 1.45; %T
vol_cy = pi*radius^2*height; %If Object is Cylinder, vol in m^3
% vol_sp = (4/3)*(pi * radius^3); %If Object is Sphere, vol in m^3

k = 0.4e-3; %additional length added to wires, to get concentric coil
%--------%--------%--------%--------%--------%--------%--------%----------
% Line along y - axis
%-%--------%--------%--------%--------%--------%--------%--------%--------
yp1_1 = -0.6e-3 - k;
yp2_1 = 0.6e-3 + k;
yn1_1 = -0.8e-3 - k;
yn2_1 = 0.8e-3 + k;
a_xp_1 = 2*g;  
a_xn_1 = -2*g;

k_yp_1 = 1/(4*pi*((a_xp_1-x)^2+z^2));
k_1yp_1 = (yp2_1-y)/((yp2_1-y)^2+(a_xp_1-x)^2+z^2)^0.5;
k_2yp_1 = (yp1_1-y)/((yp1_1-y)^2+(a_xp_1-x)^2+z^2)^0.5;

k_1yp_3 = (yp2_1-y)/((yp2_1-y)^2+(a_xp_1-x)^2+z^2)^1.5;
k_2yp_3 = (yp1_1-y)/((yp1_1-y)^2+(a_xp_1-x)^2+z^2)^1.5;

k_yn_1 = 1/(4*pi*((a_xn_1-x)^2+z^2));
k_1yn_1 = (yn2_1-y)/((yn2_1-y)^2+(a_xn_1-x)^2+z^2)^0.5;
k_2yn_1 = (yn1_1-y)/((yn1_1-y)^2+(a_xn_1-x)^2+z^2)^0.5;

k_1yn_3 = (yn2_1-y)/((yn2_1-y)^2+(a_xn_1-x)^2+z^2)^1.5;
k_2yn_3 = (yn1_1-y)/((yn1_1-y)^2+(a_xn_1-x)^2+z^2)^1.5;

hyp_x_1 = -(z*k_yp_1*(a_xp_1-x))*I*m0;
hyp_x1_1 = (k_yp_1*(k_1yp_1 - k_2yp_1))*2*4*pi;
hyp_x2_1 = k_1yp_3 - k_2yp_3;
dBxp_1_dx = hyp_x_1*(hyp_x1_1 + hyp_x2_1);

hyp_z_1 = (k_yp_1)*I*m0;
hyp_z1_1 = (k_1yp_1 - k_2yp_1)*(-1);
hyp_z2_1 = (k_yp_1*(k_1yp_1 - k_2yp_1)*(z^2))*4*pi*2;
hyp_z3_1 = (k_1yp_3 - k_2yp_3)*(z^2);
dBxp_1_dz = hyp_z_1*(hyp_z1_1 + hyp_z2_1 + hyp_z3_1);

hyn_x_1 = -(z*k_yn_1*(a_xn_1-x))*I*m0*(-1);
hyn_x1_1 = (k_yn_1*(k_1yn_1 - k_2yn_1))*2*4*pi;
hyn_x2_1 = k_1yn_3 - k_2yn_3;
dBxn_1_dx = hyn_x_1*(hyn_x1_1 + hyn_x2_1);

hyn_z_1 = (k_yn_1)*I*m0*(-1);
hyn_z1_1 = (k_1yn_1 - k_2yn_1)*(-1);
hyn_z2_1 = (k_yn_1*(k_1yn_1 - k_2yn_1)*(z^2))*4*pi*2;
hyn_z3_1 = (k_1yn_3 - k_2yn_3)*(z^2);
dBxn_1_dz = hyn_z_1*(hyn_z1_1 + hyn_z2_1 + hyn_z3_1);

%--------%--------%--------%--------%--------%--------%--------%----------
% Line along x - axis
%-%--------%--------%--------%--------%a--------%--------%--------%--------
xp1_1 = -0.8e-3 - k;
xp2_1 = 0.8e-3 + k;
xn1_1 = -1e-3 - k;
xn2_1 = 1e-3 + k;
a_yp_1 = 1.075e-3;          %Distance of coil from (0,0)
a_yn_1 = -1.075e-3;

k_xp_1 = 1/(4*pi*((a_yp_1-y)^2+z^2));
k_1xp_1 = (xp2_1-x)/((xp2_1-x)^2+(a_yp_1-y)^2+z^2)^0.5;
k_2xp_1 = (xp1_1-x)/((xp1_1-x)^2+(a_yp_1-y)^2+z^2)^0.5;

k_1xp_3 = (xp2_1-x)/((xp2_1-x)^2+(a_yp_1-y)^2+z^2)^1.5;
k_2xp_3 = (xp1_1-x)/((xp1_1-x)^2+(a_yp_1-y)^2+z^2)^1.5;

k_xn_1 = 1/(4*pi*((a_yn_1-y)^2+z^2));
k_1xn_1 = (xn2_1-x)/((xn2_1-x)^2+(a_yn_1-y)^2+z^2)^0.5;
k_2xn_1 = (xn1_1-x)/((xn1_1-x)^2+(a_yn_1-y)^2+z^2)^0.5;



k_1xn_3 = (xn2_1-x)/((xn2_1-x)^2+(a_yn_1-y)^2+z^2)^1.5;
k_2xn_3 = (xn1_1-x)/((xn1_1-x)^2+(a_yn_1-y)^2+z^2)^1.5;

hxp_x_1 = -(z*k_xp_1*(a_yp_1-y))*I*m0;
hxp_x1_1 = (k_xp_1*(k_1xp_1 - k_2xp_1))*2*4*pi;
hxp_x2_1 = k_1xp_3 - k_2xp_3;
dByp_1_dy = hxp_x_1*(hxp_x1_1 + hxp_x2_1);

hxp_z_1 = (k_xp_1)*I*m0;
hxp_z1_1 = (k_1xp_1 - k_2xp_1)*(-1);
hxp_z2_1 = (k_xp_1*(k_1xp_1 - k_2xp_1)*(z^2))*4*pi*2;
hxp_z3_1 = (k_1xp_3 - k_2xp_3)*(z^2);
dByp_1_dz = hxp_z_1*(hxp_z1_1 + hxp_z2_1 + hxp_z3_1);

hxn_x_1 = -(z*k_xn_1*(a_yn_1-y))*I*m0*(-1);
hxn_x1_1 = (k_xn_1*(k_1xn_1 - k_2xn_1))*2*4*pi;
hxn_x2_1 = k_1xn_3 - k_2xn_3;
dByn_1_dy = hxn_x_1*(hxn_x1_1 + hxn_x2_1);

hxn_z_1 = (k_xn_1)*I*m0*(-1);
hxn_z1_1 = (k_1xn_1 - k_2xn_1)*(-1);
hxn_z2_1 = (k_xn_1*(k_1xn_1 - k_2xn_1)*(z^2))*4*pi*2;
hxn_z3_1 = (k_1xn_3 - k_2xn_3)*(z^2);
dByn_1_dz = hxn_z_1*(hxn_z1_1 + hxn_z2_1 + hxn_z3_1);

F_xx_2 = vol_cy * Magentization* (dBxp_1_dx + dBxn_1_dx)/m0;
F_xz_2 = vol_cy * Magentization* (dBxp_1_dz + dBxn_1_dz)/m0;
F_yy_2 = vol_cy * Magentization* (dByp_1_dy + dByn_1_dy)/m0;
F_yz_2 = vol_cy * Magentization* (dByp_1_dz + dByn_1_dz)/m0;
end

== matlab function Coil/Outer_5_Coils/Square-10/Square - 10 ==
  data: x input; F_xx_10 output; F_xz_10 output; y input; z input; I input; F_yy_10 output; F_yz_10 output
function [F_xx_10, F_xz_10, F_yy_10, F_yz_10] = force(x, y, z, I)

g = 412e-6;     %Coil spacing
m0 = 4*pi*1e-7;
radius = 3e-3;%m
height = 1e-3;%m
Magentization = 1.45; %T
vol_cy = pi*radius^2*height; %If Object is Cylinder, vol in m^3
% vol_sp = (4/3)*(pi * radius^3); %If Object is Sphere, vol in m^3

k = 0.4e-3; %additional length added to wires, to get concentric coil
%--------%--------%--------%--------%--------%--------%--------%----------
% Line along y - axis
%-%--------%--------%--------%--------%--------%--------%--------%--------
yp1_1 = -0.6e-3 - 9*k;
yp2_1 = 0.6e-3 + 9*k;
yn1_1 = -0.8e-3 - 9*k;
yn2_1 = 0.8e-3 + 9*k;
a_xp_1 = 10*g;  
a_xn_1 = -10*g;

k_yp_1 = 1/(4*pi*((a_xp_1-x)^2+z^2));
k_1yp_1 = (yp2_1-y)/((yp2_1-y)^2+(a_xp_1-x)^2+z^2)^0.5;
k_2yp_1 = (yp1_1-y)/((yp1_1-y)^2+(a_xp_1-x)^2+z^2)^0.5;

k_1yp_3 = (yp2_1-y)/((yp2_1-y)^2+(a_xp_1-x)^2+z^2)^1.5;
k_2yp_3 = (yp1_1-y)/((yp1_1-y)^2+(a_xp_1-x)^2+z^2)^1.5;

k_yn_1 = 1/(4*pi*((a_xn_1-x)^2+z^2));
k_1yn_1 = (yn2_1-y)/((yn2_1-y)^2+(a_xn_1-x)^2+z^2)^0.5;
k_2yn_1 = (yn1_1-y)/((yn1_1-y)^2+(a_xn_1-x)^2+z^2)^0.5;

k_1yn_3 = (yn2_1-y)/((yn2_1-y)^2+(a_xn_1-x)^2+z^2)^1.5;
k_2yn_3 = (yn1_1-y)/((yn1_1-y)^2+(a_xn_1-x)^2+z^2)^1.5;

hyp_x_1 = -(z*k_yp_1*(a_xp_1-x))*I*m0;
hyp_x1_1 = (k_yp_1*(k_1yp_1 - k_2yp_1))*2*4*pi;
hyp_x2_1 = k_1yp_3 - k_2yp_3;
dBxp_1_dx = hyp_x_1*(hyp_x1_1 + hyp_x2_1);

hyp_z_1 = (k_yp_1)*I*m0;
hyp_z1_1 = (k_1yp_1 - k_2yp_1)*(-1);
hyp_z2_1 = (k_yp_1*(k_1yp_1 - k_2yp_1)*(z^2))*4*pi*2;
hyp_z3_1 = (k_1yp_3 - k_2yp_3)*(z^2);
dBxp_1_dz = hyp_z_1*(hyp_z1_1 + hyp_z2_1 + hyp_z3_1);

hyn_x_1 = -(z*k_yn_1*(a_xn_1-x))*I*m0*(-1);
hyn_x1_1 = (k_yn_1*(k_1yn_1 - k_2yn_1))*2*4*pi;
hyn_x2_1 = k_1yn_3 - k_2yn_3;
dBxn_1_dx = hyn_x_1*(hyn_x1_1 + hyn_x2_1);

hyn_z_1 = (k_yn_1)*I*m0*(-1);
hyn_z1_1 = (k_1yn_1 - k_2yn_1)*(-1);
hyn_z2_1 = (k_yn_1*(k_1yn_1 - k_2yn_1)*(z^2))*4*pi*2;
hyn_z3_1 = (k_1yn_3 - k_2yn_3)*(z^2);
dBxn_1_dz = hyn_z_1*(hyn_z1_1 + hyn_z2_1 + hyn_z3_1);

%--------%--------%--------%--------%--------%--------%--------%----------
% Line along x - axis
%-%--------%--------%--------%--------%a--------%--------%--------%--------
xp1_1 = -0.8e-3 - 9*k;
xp2_1 = 0.8e-3 + 9*k;
xn1_1 = -1e-3 - 9*k;
xn2_1 = 1e-3 + 9*k;
a_yp_1 = 4.275e-3;          %Distance of coil from (0,0)
a_yn_1 = -4.275e-3;

k_xp_1 = 1/(4*pi*((a_yp_1-y)^2+z^2));
k_1xp_1 = (xp2_1-x)/((xp2_1-x)^2+(a_yp_1-y)^2+z^2)^0.5;
k_2xp_1 = (xp1_1-x)/((xp1_1-x)^2+(a_yp_1-y)^2+z^2)^0.5;

k_xn_1 = 1/(4*pi*((a_yn_1-y)^2+z^2));
k_1xn_1 = (xn2_1-x)/((xn2_1-x)^2+(a_yn_1-y)^2+z^2)^0.5;
k_2xn_1 = (xn1_1-x)/((xn1_1-x)^2+(a_yn_1-y)^2+z^2)^0.5;

k_1xp_3 = (xp2_1-x)/((xp2_1-x)^2+(a_yp_1-y)^2+z^2)^1.5;
k_2xp_3 = (xp1_1-x)/((xp1_1-x)^2+(a_yp_1-y)^2+z^2)^1.5;

k_1xn_3 = (xn2_1-x)/((xn2_1-x)^2+(a_yn_1-y)^2+z^2)^1.5;
k_2xn_3 = (xn1_1-x)/((xn1_1-x)^2+(a_yn_1-y)^2+z^2)^1.5;

hxp_x_1 = -(z*k_xp_1*(a_yp_1-y))*I*m0;
hxp_x1_1 = (k_xp_1*(k_1xp_1 - k_2xp_1))*2*4*pi;
hxp_x2_1 = k_1xp_3 - k_2xp_3;
dByp_1_dy = hxp_x_1*(hxp_x1_1 + hxp_x2_1);

hxp_z_1 = (k_xp_1)*I*m0;
hxp_z1_1 = (k_1xp_1 - k_2xp_1)*(-1);
hxp_z2_1 = (k_xp_1*(k_1xp_1 - k_2xp_1)*(z^2))*4*pi*2;
hxp_z3_1 = (k_1xp_3 - k_2xp_3)*(z^2);
dByp_1_dz = hxp_z_1*(hxp_z1_1 + hxp_z2_1 + hxp_z3_1);

hxn_x_1 = -(z*k_xn_1*(a_yn_1-y))*I*m0*(-1);
hxn_x1_1 = (k_xn_1*(k_1xn_1 - k_2xn_1))*2*4*pi;
hxn_x2_1 = k_1xn_3 - k_2xn_3;
dByn_1_dy = hxn_x_1*(hxn_x1_1 + hxn_x2_1);

hxn_z_1 = (k_xn_1)*I*m0*(-1);
hxn_z1_1 = (k_1xn_1 - k_2xn_1)*(-1);
hxn_z2_1 = (k_xn_1*(k_1xn_1 - k_2xn_1)*(z^2))*4*pi*2;
hxn_z3_1 = (k_1xn_3 - k_2xn_3)*(z^2);
dByn_1_dz = hxn_z_1*(hxn_z1_1 + hxn_z2_1 + hxn_z3_1);

F_xx_10 = vol_cy * Magentization* (dBxp_1_dx + dBxn_1_dx)/m0;
F_xz_10 = vol_cy * Magentization* (dBxp_1_dz + dBxn_1_dz)/m0;
F_yy_10 = vol_cy * Magentization* (dByp_1_dy + dByn_1_dy)/m0;
F_yz_10 = vol_cy * Magentization* (dByp_1_dz + dByn_1_dz)/m0;
end

== matlab function Coil/Inner_5_coils/Square-1/Square - 1 ==
  data: x input; F_xx_1 output; F_xz_1 output; y input; z input; I input; F_yy_1 output; F_yz_1 output
function [F_xx_1, F_xz_1, F_yy_1, F_yz_1] = force(x, y, z, I)

g = 520e-6;     %Coil spacing from start of one coil to another
m0 = 4*pi*1e-7;
radius = 3e-3;%m
height = 1e-3;%m
Magentization = 1.45; %T
vol_cy = pi*radius^2*height; %If Object is Cylinder, vol in m^3
% vol_sp = (4/3)*(pi * radius^3); %If Object is Sphere, vol in m^3

k = 0.4e-3; %additional length added to wires, to get concentric coil
%--------%--------%--------%--------%--------%--------%--------%----------
% Line along y - axis
%-%--------%--------%--------%--------%--------%--------%--------%--------
yp1_1 = -0.6e-3;
yp2_1 = 0.6e-3;
yn1_1 = -0.8e-3;
yn2_1 = 0.8e-3;
a_xp_1 = g;  
a_xn_1 = -g;

k_yp_1 = 1/(4*pi*((a_xp_1-x)^2+z^2));
k_1yp_1 = (yp2_1-y)/((yp2_1-y)^2+(a_xp_1-x)^2+z^2)^0.5;
k_2yp_1 = (yp1_1-y)/((yp1_1-y)^2+(a_xp_1-x)^2+z^2)^0.5;

k_1yp_3 = (yp2_1-y)/((yp2_1-y)^2+(a_xp_1-x)^2+z^2)^1.5;
k_2yp_3 = (yp1_1-y)/((yp1_1-y)^2+(a_xp_1-x)^2+z^2)^1.5;

k_yn_1 = 1/(4*pi*((a_xn_1-x)^2+z^2));
k_1yn_1 = (yn2_1-y)/((yn2_1-y)^2+(a_xn_1-x)^2+z^2)^0.5;
k_2yn_1 = (yn1_1-y)/((yn1_1-y)^2+(a_xn_1-x)^2+z^2)^0.5;

k_1yn_3 = (yn2_1-y)/((yn2_1-y)^2+(a_xn_1-x)^2+z^2)^1.5;
k_2yn_3 = (yn1_1-y)/((yn1_1-y)^2+(a_xn_1-x)^2+z^2)^1.5;

hyp_x_1 = -(z*k_yp_1*(a_xp_1-x))*I*m0;
hyp_x1_1 = (k_yp_1*(k_1yp_1 - k_2yp_1))*2*4*pi;
hyp_x2_1 = k_1yp_3 - k_2yp_3;
dBxp_1_dx = hyp_x_1*(hyp_x1_1 + hyp_x2_1);

hyp_z_1 = (k_yp_1)*I*m0;
hyp_z1_1 = (k_1yp_1 - k_2yp_1)*(-1);
hyp_z2_1 = (k_yp_1*(k_1yp_1 - k_2yp_1)*(z^2))*4*pi*2;
hyp_z3_1 = (k_1yp_3 - k_2yp_3)*(z^2);
dBxp_1_dz = hyp_z_1*(hyp_z1_1 + hyp_z2_1 + hyp_z3_1);

hyn_x_1 = -(z*k_yn_1*(a_xn_1-x))*I*m0*(-1);
hyn_x1_1 = (k_yn_1*(k_1yn_1 - k_2yn_1))*2*4*pi;
hyn_x2_1 = k_1yn_3 - k_2yn_3;
dBxn_1_dx = hyn_x_1*(hyn_x1_1 + hyn_x2_1);

hyn_z_1 = (k_yn_1)*I*m0*(-1);
hyn_z1_1 = (k_1yn_1 - k_2yn_1)*(-1);
hyn_z2_1 = (k_yn_1*(k_1yn_1 - k_2yn_1)*(z^2))*4*pi*2;
hyn_z3_1 = (k_1yn_3 - k_2yn_3)*(z^2);
dBxn_1_dz = hyn_z_1*(hyn_z1_1 + hyn_z2_1 + hyn_z3_1);

%--------%--------%--------%--------%--------%--------%--------%----------
% Line along x - axis
%-%--------%--------%--------%--------%a--------%--------%--------%--------
xp1_1 = -0.8e-3;
xp2_1 = 0.8e-3;
xn1_1 = -1e-3;
xn2_1 = 1e-3;
a_yp_1 = 0.675e-3;          %Distance of coil from (0,0)
a_yn_1 = -0.675e-3;

k_xp_1 = 1/(4*pi*((a_yp_1-y)^2+z^2));
k_1xp_1 = (xp2_1-x)/((xp2_1-x)^2+(a_yp_1-y)^2+z^2)^0.5;
k_2xp_1 = (xp1_1-x)/((xp1_1-x)^2+(a_yp_1-y)^2+z^2)^0.5;

k_xn_1 = 1/(4*pi*((a_yn_1-y)^2+z^2));
k_1xn_1 = (xn2_1-x)/((xn2_1-x)^2+(a_yn_1-y)^2+z^2)^0.5;
k_2xn_1 = (xn1_1-x)/((xn1_1-x)^2+(a_yn_1-y)^2+z^2)^0.5;

k_1xp_3 = (xp2_1-x)/((xp2_1-x)^2+(a_yp_1-y)^2+z^2)^1.5;
k_2xp_3 = (xp1_1-x)/((xp1_1-x)^2+(a_yp_1-y)^2+z^2)^1.5;

k_1xn_3 = (xn2_1-x)/((xn2_1-x)^2+(a_yn_1-y)^2+z^2)^1.5;
k_2xn_3 = (xn1_1-x)/((xn1_1-x)^2+(a_yn_1-y)^2+z^2)^1.5;

hxp_x_1 = -(z*k_xp_1*(a_yp_1-y))*I*m0;
hxp_x1_1 = (k_xp_1*(k_1xp_1 - k_2xp_1))*2*4*pi;
hxp_x2_1 = k_1xp_3 - k_2xp_3;
dByp_1_dy = hxp_x_1*(hxp_x1_1 + hxp_x2_1);

hxp_z_1 = (k_xp_1)*I*m0;
hxp_z1_1 = (k_1xp_1 - k_2xp_1)*(-1);
hxp_z2_1 = (k_xp_1*(k_1xp_1 - k_2xp_1)*(z^2))*4*pi*2;
hxp_z3_1 = (k_1xp_3 - k_2xp_3)*(z^2);
dByp_1_dz = hxp_z_1*(hxp_z1_1 + hxp_z2_1 + hxp_z3_1);

hxn_x_1 = -(z*k_xn_1*(a_yn_1-y))*I*m0*(-1);
hxn_x1_1 = (k_xn_1*(k_1xn_1 - k_2xn_1))*2*4*pi;
hxn_x2_1 = k_1xn_3 - k_2xn_3;
dByn_1_dy = hxn_x_1*(hxn_x1_1 + hxn_x2_1);

hxn_z_1 = (k_xn_1)*I*m0*(-1);
hxn_z1_1 = (k_1xn_1 - k_2xn_1)*(-1);
hxn_z2_1 = (k_xn_1*(k_1xn_1 - k_2xn_1)*(z^2))*4*pi*2;
hxn_z3_1 = (k_1xn_3 - k_2xn_3)*(z^2);
dByn_1_dz = hxn_z_1*(hxn_z1_1 + hxn_z2_1 + hxn_z3_1);

F_xx_1 = vol_cy * Magentization* (dBxp_1_dx + dBxn_1_dx)/m0;
F_xz_1 = vol_cy * Magentization* (dBxp_1_dz + dBxn_1_dz)/m0;
F_yy_1 = vol_cy * Magentization* (dByp_1_dy + dByn_1_dy)/m0;
F_yz_1 = vol_cy * Magentization* (dByp_1_dz + dByn_1_dz)/m0;
end

== matlab function Coil/Inner_5_coils/Square-3/Square - 3 ==
  data: x input; F_xx_3 output; F_xz_3 output; y input; z input; I input; F_yy_3 output; F_yz_3 output
function [F_xx_3, F_xz_3, F_yy_3, F_yz_3] = force(x, y, z, I)

g = 440e-6;     %Coil spacing
m0 = 4*pi*1e-7;
radius = 3e-3;%m
height = 1e-3;%m
Magentization = 1.45; %T
vol_cy = pi*radius^2*height; %If Object is Cylinder, vol in m^3
% vol_sp = (4/3)*(pi * radius^3); %If Object is Sphere, vol in m^3

k = 0.4e-3; %additional length added to wires, to get concentric coil
%--------%--------%--------%--------%--------%--------%--------%----------
% Line along y - axis
%-%--------%--------%--------%--------%--------%--------%--------%--------
yp1_1 = -0.6e-3 - 2*k;
yp2_1 = 0.6e-3 + 2*k;
yn1_1 = -0.8e-3 - 2*k;
yn2_1 = 0.8e-3 + 2*k;
a_xp_1 = 3*g;  
a_xn_1 = -3*g;

k_yp_1 = 1/(4*pi*((a_xp_1-x)^2+z^2));
k_1yp_1 = (yp2_1-y)/((yp2_1-y)^2+(a_xp_1-x)^2+z^2)^0.5;
k_2yp_1 = (yp1_1-y)/((yp1_1-y)^2+(a_xp_1-x)^2+z^2)^0.5;

k_1yp_3 = (yp2_1-y)/((yp2_1-y)^2+(a_xp_1-x)^2+z^2)^1.5;
k_2yp_3 = (yp1_1-y)/((yp1_1-y)^2+(a_xp_1-x)^2+z^2)^1.5;

k_yn_1 = 1/(4*pi*((a_xn_1-x)^2+z^2));
k_1yn_1 = (yn2_1-y)/((yn2_1-y)^2+(a_xn_1-x)^2+z^2)^0.5;
k_2yn_1 = (yn1_1-y)/((yn1_1-y)^2+(a_xn_1-x)^2+z^2)^0.5;

k_1yn_3 = (yn2_1-y)/((yn2_1-y)^2+(a_xn_1-x)^2+z^2)^1.5;
k_2yn_3 = (yn1_1-y)/((yn1_1-y)^2+(a_xn_1-x)^2+z^2)^1.5;



hyp_x_1 = -(z*k_yp_1*(a_xp_1-x))*I*m0;
hyp_x1_1 = (k_yp_1*(k_1yp_1 - k_2yp_1))*2*4*pi;
hyp_x2_1 = k_1yp_3 - k_2yp_3;
dBxp_1_dx = hyp_x_1*(hyp_x1_1 + hyp_x2_1);

hyp_z_1 = (k_yp_1)*I*m0;
hyp_z1_1 = (k_1yp_1 - k_2yp_1)*(-1);
hyp_z2_1 = (k_yp_1*(k_1yp_1 - k_2yp_1)*(z^2))*4*pi*2;
hyp_z3_1 = (k_1yp_3 - k_2yp_3)*(z^2);
dBxp_1_dz = hyp_z_1*(hyp_z1_1 + hyp_z2_1 + hyp_z3_1);

hyn_x_1 = -(z*k_yn_1*(a_xn_1-x))*I*m0*(-1);
hyn_x1_1 = (k_yn_1*(k_1yn_1 - k_2yn_1))*2*4*pi;
hyn_x2_1 = k_1yn_3 - k_2yn_3;
dBxn_1_dx = hyn_x_1*(hyn_x1_1 + hyn_x2_1);

hyn_z_1 = (k_yn_1)*I*m0*(-1);
hyn_z1_1 = (k_1yn_1 - k_2yn_1)*(-1);
hyn_z2_1 = (k_yn_1*(k_1yn_1 - k_2yn_1)*(z^2))*4*pi*2;
hyn_z3_1 = (k_1yn_3 - k_2yn_3)*(z^2);
dBxn_1_dz = hyn_z_1*(hyn_z1_1 + hyn_z2_1 + hyn_z3_1);

%--------%--------%--------%--------%--------%--------%--------%----------
% Line along x - axis
%-%--------%--------%--------%--------%a--------%--------%--------%--------
xp1_1 = -0.8e-3 - 2*k;
xp2_1 = 0.8e-3 + 2*k;
xn1_1 = -1e-3 - 2*k;
xn2_1 = 1e-3 + 2*k;
a_yp_1 = 1.475e-3;          %Distance of coil from (0,0)
a_yn_1 = -1.475e-3;

k_xp_1 = 1/(4*pi*((a_yp_1-y)^2+z^2));
k_1xp_1 = (xp2_1-x)/((xp2_1-x)^2+(a_yp_1-y)^2+z^2)^0.5;
k_2xp_1 = (xp1_1-x)/((xp1_1-x)^2+(a_yp_1-y)^2+z^2)^0.5;

k_xn_1 = 1/(4*pi*((a_yn_1-y)^2+z^2));
k_1xn_1 = (xn2_1-x)/((xn2_1-x)^2+(a_yn_1-y)^2+z^2)^0.5;
k_2xn_1 = (xn1_1-x)/((xn1_1-x)^2+(a_yn_1-y)^2+z^2)^0.5;

k_1xp_3 = (xp2_1-x)/((xp2_1-x)^2+(a_yp_1-y)^2+z^2)^1.5;
k_2xp_3 = (xp1_1-x)/((xp1_1-x)^2+(a_yp_1-y)^2+z^2)^1.5;

k_1xn_3 = (xn2_1-x)/((xn2_1-x)^2+(a_yn_1-y)^2+z^2)^1.5;
k_2xn_3 = (xn1_1-x)/((xn1_1-x)^2+(a_yn_1-y)^2+z^2)^1.5;

hxp_x_1 = -(z*k_xp_1*(a_yp_1-y))*I*m0;
hxp_x1_1 = (k_xp_1*(k_1xp_1 - k_2xp_1))*2*4*pi;
hxp_x2_1 = k_1xp_3 - k_2xp_3;
dByp_1_dy = hxp_x_1*(hxp_x1_1 + hxp_x2_1);

hxp_z_1 = (k_xp_1)*I*m0;
hxp_z1_1 = (k_1xp_1 - k_2xp_1)*(-1);
hxp_z2_1 = (k_xp_1*(k_1xp_1 - k_2xp_1)*(z^2))*4*pi*2;
hxp_z3_1 = (k_1xp_3 - k_2xp_3)*(z^2);
dByp_1_dz = hxp_z_1*(hxp_z1_1 + hxp_z2_1 + hxp_z3_1);

hxn_x_1 = -(z*k_xn_1*(a_yn_1-y))*I*m0*(-1);
hxn_x1_1 = (k_xn_1*(k_1xn_1 - k_2xn_1))*2*4*pi;
hxn_x2_1 = k_1xn_3 - k_2xn_3;
dByn_1_dy = hxn_x_1*(hxn_x1_1 + hxn_x2_1);

hxn_z_1 = (k_xn_1)*I*m0*(-1);
hxn_z1_1 = (k_1xn_1 - k_2xn_1)*(-1);
hxn_z2_1 = (k_xn_1*(k_1xn_1 - k_2xn_1)*(z^2))*4*pi*2;
hxn_z3_1 = (k_1xn_3 - k_2xn_3)*(z^2);
dByn_1_dz = hxn_z_1*(hxn_z1_1 + hxn_z2_1 + hxn_z3_1);

F_xx_3 = vol_cy * Magentization* (dBxp_1_dx + dBxn_1_dx)/m0;
F_xz_3 = vol_cy * Magentization* (dBxp_1_dz + dBxn_1_dz)/m0;
F_yy_3 = vol_cy * Magentization* (dByp_1_dy + dByn_1_dy)/m0;
F_yz_3 = vol_cy * Magentization* (dByp_1_dz + dByn_1_dz)/m0;
end

== matlab function Coil/Inner_5_coils/Square-4/Square - 4 ==
  data: x input; F_xx_4 output; F_xz_4 output; y input; z input; I input; F_yy_4 output; F_yz_4 output
function [F_xx_4, F_xz_4, F_yy_4, F_yz_4] = force(x, y, z, I)

g = 430e-6;     %Coil spacing
m0 = 4*pi*1e-7;
radius = 3e-3;%m
height = 1e-3;%m
Magentization = 1.45; %T
vol_cy = pi*radius^2*height; %If Object is Cylinder, vol in m^3
% vol_sp = (4/3)*(pi * radius^3); %If Object is Sphere, vol in m^3

k = 0.4e-3; %additional length added to wires, to get concentric coil
%--------%--------%--------%--------%--------%--------%--------%----------
% Line along y - axis
%-%--------%--------%--------%--------%--------%--------%--------%--------
yp1_1 = -0.6e-3 - 3*k;
yp2_1 = 0.6e-3 + 3*k;
yn1_1 = -0.8e-3 - 3*k;
yn2_1 = 0.8e-3 + 3*k;
a_xp_1 = 4*g;  
a_xn_1 = -4*g;

k_yp_1 = 1/(4*pi*((a_xp_1-x)^2+z^2));
k_1yp_1 = (yp2_1-y)/((yp2_1-y)^2+(a_xp_1-x)^2+z^2)^0.5;
k_2yp_1 = (yp1_1-y)/((yp1_1-y)^2+(a_xp_1-x)^2+z^2)^0.5;

k_1yp_3 = (yp2_1-y)/((yp2_1-y)^2+(a_xp_1-x)^2+z^2)^1.5;
k_2yp_3 = (yp1_1-y)/((yp1_1-y)^2+(a_xp_1-x)^2+z^2)^1.5;

k_yn_1 = 1/(4*pi*((a_xn_1-x)^2+z^2));
k_1yn_1 = (yn2_1-y)/((yn2_1-y)^2+(a_xn_1-x)^2+z^2)^0.5;
k_2yn_1 = (yn1_1-y)/((yn1_1-y)^2+(a_xn_1-x)^2+z^2)^0.5;

k_1yn_3 = (yn2_1-y)/((yn2_1-y)^2+(a_xn_1-x)^2+z^2)^1.5;
k_2yn_3 = (yn1_1-y)/((yn1_1-y)^2+(a_xn_1-x)^2+z^2)^1.5;

hyp_x_1 = -(z*k_yp_1*(a_xp_1-x))*I*m0;
hyp_x1_1 = (k_yp_1*(k_1yp_1 - k_2yp_1))*2*4*pi;
hyp_x2_1 = k_1yp_3 - k_2yp_3;
dBxp_1_dx = hyp_x_1*(hyp_x1_1 + hyp_x2_1);

hyp_z_1 = (k_yp_1)*I*m0;
hyp_z1_1 = (k_1yp_1 - k_2yp_1)*(-1);
hyp_z2_1 = (k_yp_1*(k_1yp_1 - k_2yp_1)*(z^2))*4*pi*2;
hyp_z3_1 = (k_1yp_3 - k_2yp_3)*(z^2);
dBxp_1_dz = hyp_z_1*(hyp_z1_1 + hyp_z2_1 + hyp_z3_1);

hyn_x_1 = -(z*k_yn_1*(a_xn_1-x))*I*m0*(-1);
hyn_x1_1 = (k_yn_1*(k_1yn_1 - k_2yn_1))*2*4*pi;
hyn_x2_1 = k_1yn_3 - k_2yn_3;
dBxn_1_dx = hyn_x_1*(hyn_x1_1 + hyn_x2_1);

hyn_z_1 = (k_yn_1)*I*m0*(-1);
hyn_z1_1 = (k_1yn_1 - k_2yn_1)*(-1);
hyn_z2_1 = (k_yn_1*(k_1yn_1 - k_2yn_1)*(z^2))*4*pi*2;
hyn_z3_1 = (k_1yn_3 - k_2yn_3)*(z^2);
dBxn_1_dz = hyn_z_1*(hyn_z1_1 + hyn_z2_1 + hyn_z3_1);

%--------%--------%--------%--------%--------%--------%--------%----------
% Line along x - axis
%-%--------%--------%--------%--------%a--------%--------%--------%--------
xp1_1 = -0.8e-3 - 3*k;
xp2_1 = 0.8e-3 + 3*k;
xn1_1 = -1e-3 - 3*k;
xn2_1 = 1e-3 + 3*k;
a_yp_1 = 1.875e-3;          %Distance of coil from (0,0)
a_yn_1 = -1.875e-3;

k_xp_1 = 1/(4*pi*((a_yp_1-y)^2+z^2));
k_1xp_1 = (xp2_1-x)/((xp2_1-x)^2+(a_yp_1-y)^2+z^2)^0.5;
k_2xp_1 = (xp1_1-x)/((xp1_1-x)^2+(a_yp_1-y)^2+z^2)^0.5;

k_xn_1 = 1/(4*pi*((a_yn_1-y)^2+z^2));
k_1xn_1 = (xn2_1-x)/((xn2_1-x)^2+(a_yn_1-y)^2+z^2)^0.5;
k_2xn_1 = (xn1_1-x)/((xn1_1-x)^2+(a_yn_1-y)^2+z^2)^0.5;

k_1xp_3 = (xp2_1-x)/((xp2_1-x)^2+(a_yp_1-y)^2+z^2)^1.5;
k_2xp_3 = (xp1_1-x)/((xp1_1-x)^2+(a_yp_1-y)^2+z^2)^1.5;

k_1xn_3 = (xn2_1-x)/((xn2_1-x)^2+(a_yn_1-y)^2+z^2)^1.5;
k_2xn_3 = (xn1_1-x)/((xn1_1-x)^2+(a_yn_1-y)^2+z^2)^1.5;

hxp_x_1 = -(z*k_xp_1*(a_yp_1-y))*I*m0;
hxp_x1_1 = (k_xp_1*(k_1xp_1 - k_2xp_1))*2*4*pi;
hxp_x2_1 = k_1xp_3 - k_2xp_3;
dByp_1_dy = hxp_x_1*(hxp_x1_1 + hxp_x2_1);

hxp_z_1 = (k_xp_1)*I*m0;
hxp_z1_1 = (k_1xp_1 - k_2xp_1)*(-1);
hxp_z2_1 = (k_xp_1*(k_1xp_1 - k_2xp_1)*(z^2))*4*pi*2;
hxp_z3_1 = (k_1xp_3 - k_2xp_3)*(z^2);
dByp_1_dz = hxp_z_1*(hxp_z1_1 + hxp_z2_1 + hxp_z3_1);

hxn_x_1 = -(z*k_xn_1*(a_yn_1-y))*I*m0*(-1);
hxn_x1_1 = (k_xn_1*(k_1xn_1 - k_2xn_1))*2*4*pi;
hxn_x2_1 = k_1xn_3 - k_2xn_3;
dByn_1_dy = hxn_x_1*(hxn_x1_1 + hxn_x2_1);

hxn_z_1 = (k_xn_1)*I*m0*(-1);
hxn_z1_1 = (k_1xn_1 - k_2xn_1)*(-1);
hxn_z2_1 = (k_xn_1*(k_1xn_1 - k_2xn_1)*(z^2))*4*pi*2;
hxn_z3_1 = (k_1xn_3 - k_2xn_3)*(z^2);
dByn_1_dz = hxn_z_1*(hxn_z1_1 + hxn_z2_1 + hxn_z3_1);

F_xx_4 = vol_cy * Magentization* (dBxp_1_dx + dBxn_1_dx)/m0;
F_xz_4 = vol_cy * Magentization* (dBxp_1_dz + dBxn_1_dz)/m0;
F_yy_4 = vol_cy * Magentization* (dByp_1_dy + dByn_1_dy)/m0;
F_yz_4 = vol_cy * Magentization* (dByp_1_dz + dByn_1_dz)/m0;
end

== matlab function Coil/Inner_5_coils/Square-5/Square - 5 ==
  data: x input; F_xx_5 output; F_xz_5 output; y input; z input; I input; F_yy_5 output; F_yz_5 output
function [F_xx_5, F_xz_5, F_yy_5, F_yz_5] = force(x, y, z, I)

g = 424e-6;     %Coil spacing
m0 = 4*pi*1e-7;
radius = 3e-3;%m
height = 1e-3;%m
Magentization = 1.45; %T
vol_cy = pi*radius^2*height; %If Object is Cylinder, vol in m^3
% vol_sp = (4/3)*(pi * radius^3); %If Object is Sphere, vol in m^3

k = 0.4e-3; %additional length added to wires, to get concentric coil
%--------%--------%--------%--------%--------%--------%--------%----------
% Line along y - axis
%-%--------%--------%--------%--------%--------%--------%--------%--------
yp1_1 = -0.6e-3 - 4*k;
yp2_1 = 0.6e-3 + 4*k;
yn1_1 = -0.8e-3 - 4*k;
yn2_1 = 0.8e-3 + 4*k;
a_xp_1 = 5*g;  
a_xn_1 = -5*g;

k_yp_1 = 1/(4*pi*((a_xp_1-x)^2+z^2));
k_1yp_1 = (yp2_1-y)/((yp2_1-y)^2+(a_xp_1-x)^2+z^2)^0.5;
k_2yp_1 = (yp1_1-y)/((yp1_1-y)^2+(a_xp_1-x)^2+z^2)^0.5;

k_1yp_3 = (yp2_1-y)/((yp2_1-y)^2+(a_xp_1-x)^2+z^2)^1.5;
k_2yp_3 = (yp1_1-y)/((yp1_1-y)^2+(a_xp_1-x)^2+z^2)^1.5;

k_yn_1 = 1/(4*pi*((a_xn_1-x)^2+z^2));
k_1yn_1 = (yn2_1-y)/((yn2_1-y)^2+(a_xn_1-x)^2+z^2)^0.5;
k_2yn_1 = (yn1_1-y)/((yn1_1-y)^2+(a_xn_1-x)^2+z^2)^0.5;

k_1yn_3 = (yn2_1-y)/((yn2_1-y)^2+(a_xn_1-x)^2+z^2)^1.5;
k_2yn_3 = (yn1_1-y)/((yn1_1-y)^2+(a_xn_1-x)^2+z^2)^1.5;

hyp_x_1 = -(z*k_yp_1*(a_xp_1-x))*I*m0;
hyp_x1_1 = (k_yp_1*(k_1yp_1 - k_2yp_1))*2*4*pi;
hyp_x2_1 = k_1yp_3 - k_2yp_3;
dBxp_1_dx = hyp_x_1*(hyp_x1_1 + hyp_x2_1);

hyp_z_1 = (k_yp_1)*I*m0;
hyp_z1_1 = (k_1yp_1 - k_2yp_1)*(-1);
hyp_z2_1 = (k_yp_1*(k_1yp_1 - k_2yp_1)*(z^2))*4*pi*2;
hyp_z3_1 = (k_1yp_3 - k_2yp_3)*(z^2);
dBxp_1_dz = hyp_z_1*(hyp_z1_1 + hyp_z2_1 + hyp_z3_1);

hyn_x_1 = -(z*k_yn_1*(a_xn_1-x))*I*m0*(-1);
hyn_x1_1 = (k_yn_1*(k_1yn_1 - k_2yn_1))*2*4*pi;
hyn_x2_1 = k_1yn_3 - k_2yn_3;
dBxn_1_dx = hyn_x_1*(hyn_x1_1 + hyn_x2_1);

hyn_z_1 = (k_yn_1)*I*m0*(-1);
hyn_z1_1 = (k_1yn_1 - k_2yn_1)*(-1);
hyn_z2_1 = (k_yn_1*(k_1yn_1 - k_2yn_1)*(z^2))*4*pi*2;
hyn_z3_1 = (k_1yn_3 - k_2yn_3)*(z^2);
dBxn_1_dz = hyn_z_1*(hyn_z1_1 + hyn_z2_1 + hyn_z3_1);

%--------%--------%--------%--------%--------%--------%--------%----------
% Line along x - axis
%-%--------%--------%--------%--------%a--------%--------%--------%--------
xp1_1 = -0.8e-3 - 4*k;
xp2_1 = 0.8e-3 + 4*k;
xn1_1 = -1e-3 - 4*k;
xn2_1 = 1e-3 + 4*k;
a_yp_1 = 2.275e-3;          %Distance of coil from (0,0)
a_yn_1 = -2.275e-3;

k_xp_1 = 1/(4*pi*((a_yp_1-y)^2+z^2));
k_1xp_1 = (xp2_1-x)/((xp2_1-x)^2+(a_yp_1-y)^2+z^2)^0.5;
k_2xp_1 = (xp1_1-x)/((xp1_1-x)^2+(a_yp_1-y)^2+z^2)^0.5;

k_xn_1 = 1/(4*pi*((a_yn_1-y)^2+z^2));
k_1xn_1 = (xn2_1-x)/((xn2_1-x)^2+(a_yn_1-y)^2+z^2)^0.5;
k_2xn_1 = (xn1_1-x)/((xn1_1-x)^2+(a_yn_1-y)^2+z^2)^0.5;

k_1xp_3 = (xp2_1-x)/((xp2_1-x)^2+(a_yp_1-y)^2+z^2)^1.5;
k_2xp_3 = (xp1_1-x)/((xp1_1-x)^2+(a_yp_1-y)^2+z^2)^1.5;

k_1xn_3 = (xn2_1-x)/((xn2_1-x)^2+(a_yn_1-y)^2+z^2)^1.5;
k_2xn_3 = (xn1_1-x)/((xn1_1-x)^2+(a_yn_1-y)^2+z^2)^1.5;

hxp_x_1 = -(z*k_xp_1*(a_yp_1-y))*I*m0;
hxp_x1_1 = (k_xp_1*(k_1xp_1 - k_2xp_1))*2*4*pi;
hxp_x2_1 = k_1xp_3 - k_2xp_3;
dByp_1_dy = hxp_x_1*(hxp_x1_1 + hxp_x2_1);

hxp_z_1 = (k_xp_1)*I*m0;
hxp_z1_1 = (k_1xp_1 - k_2xp_1)*(-1);
hxp_z2_1 = (k_xp_1*(k_1xp_1 - k_2xp_1)*(z^2))*4*pi*2;
hxp_z3_1 = (k_1xp_3 - k_2xp_3)*(z^2);
dByp_1_dz = hxp_z_1*(hxp_z1_1 + hxp_z2_1 + hxp_z3_1);

hxn_x_1 = -(z*k_xn_1*(a_yn_1-y))*I*m0*(-1);
hxn_x1_1 = (k_xn_1*(k_1xn_1 - k_2xn_1))*2*4*pi;
hxn_x2_1 = k_1xn_3 - k_2xn_3;
dByn_1_dy = hxn_x_1*(hxn_x1_1 + hxn_x2_1);

hxn_z_1 = (k_xn_1)*I*m0*(-1);
hxn_z1_1 = (k_1xn_1 - k_2xn_1)*(-1);
hxn_z2_1 = (k_xn_1*(k_1xn_1 - k_2xn_1)*(z^2))*4*pi*2;
hxn_z3_1 = (k_1xn_3 - k_2xn_3)*(z^2);
dByn_1_dz = hxn_z_1*(hxn_z1_1 + hxn_z2_1 + hxn_z3_1);

F_xx_5 = vol_cy * Magentization* (dBxp_1_dx + dBxn_1_dx)/m0;
F_xz_5 = vol_cy * Magentization* (dBxp_1_dz + dBxn_1_dz)/m0;
F_yy_5 = vol_cy * Magentization* (dByp_1_dy + dByn_1_dy)/m0;
F_yz_5 = vol_cy * Magentization* (dByp_1_dz + dByn_1_dz)/m0;
end

== matlab function Coil/Outer_5_Coils/Square-6/Square - 6 ==
  data: x input; F_xx_6 output; F_xz_6 output; y input; z input; I input; F_yy_6 output; F_yz_6 output
function [F_xx_6, F_xz_6, F_yy_6, F_yz_6] = force(x, y, z, I)

g = 420e-6;     %Coil spacing
m0 = 4*pi*1e-7;
radius = 3e-3;%m
height = 1e-3;%m
Magentization = 1.45; %T
vol_cy = pi*radius^2*height; %If Object is Cylinder, vol in m^3
% vol_sp = (4/3)*(pi * radius^3); %If Object is Sphere, vol in m^3

k = 0.4e-3; %additional length added to wires, to get concentric coil
%--------%--------%--------%--------%--------%--------%--------%----------
% Line along y - axis
%-%--------%--------%--------%--------%--------%--------%--------%--------
yp1_1 = -0.6e-3 - 5*k;
yp2_1 = 0.6e-3 + 5*k;
yn1_1 = -0.8e-3 - 5*k;
yn2_1 = 0.8e-3 + 5*k;
a_xp_1 = 6*g;  
a_xn_1 = -6*g;

k_yp_1 = 1/(4*pi*((a_xp_1-x)^2+z^2));
k_1yp_1 = (yp2_1-y)/((yp2_1-y)^2+(a_xp_1-x)^2+z^2)^0.5;
k_2yp_1 = (yp1_1-y)/((yp1_1-y)^2+(a_xp_1-x)^2+z^2)^0.5;

k_1yp_3 = (yp2_1-y)/((yp2_1-y)^2+(a_xp_1-x)^2+z^2)^1.5;
k_2yp_3 = (yp1_1-y)/((yp1_1-y)^2+(a_xp_1-x)^2+z^2)^1.5;

k_yn_1 = 1/(4*pi*((a_xn_1-x)^2+z^2));
k_1yn_1 = (yn2_1-y)/((yn2_1-y)^2+(a_xn_1-x)^2+z^2)^0.5;
k_2yn_1 = (yn1_1-y)/((yn1_1-y)^2+(a_xn_1-x)^2+z^2)^0.5;

k_1yn_3 = (yn2_1-y)/((yn2_1-y)^2+(a_xn_1-x)^2+z^2)^1.5;
k_2yn_3 = (yn1_1-y)/((yn1_1-y)^2+(a_xn_1-x)^2+z^2)^1.5;

hyp_x_1 = -(z*k_yp_1*(a_xp_1-x))*I*m0;
hyp_x1_1 = (k_yp_1*(k_1yp_1 - k_2yp_1))*2*4*pi;
hyp_x2_1 = k_1yp_3 - k_2yp_3;
dBxp_1_dx = hyp_x_1*(hyp_x1_1 + hyp_x2_1);

hyp_z_1 = (k_yp_1)*I*m0;
hyp_z1_1 = (k_1yp_1 - k_2yp_1)*(-1);
hyp_z2_1 = (k_yp_1*(k_1yp_1 - k_2yp_1)*(z^2))*4*pi*2;
hyp_z3_1 = (k_1yp_3 - k_2yp_3)*(z^2);
dBxp_1_dz = hyp_z_1*(hyp_z1_1 + hyp_z2_1 + hyp_z3_1);

hyn_x_1 = -(z*k_yn_1*(a_xn_1-x))*I*m0*(-1);
hyn_x1_1 = (k_yn_1*(k_1yn_1 - k_2yn_1))*2*4*pi;
hyn_x2_1 = k_1yn_3 - k_2yn_3;
dBxn_1_dx = hyn_x_1*(hyn_x1_1 + hyn_x2_1);

hyn_z_1 = (k_yn_1)*I*m0*(-1);
hyn_z1_1 = (k_1yn_1 - k_2yn_1)*(-1);
hyn_z2_1 = (k_yn_1*(k_1yn_1 - k_2yn_1)*(z^2))*4*pi*2;
hyn_z3_1 = (k_1yn_3 - k_2yn_3)*(z^2);
dBxn_1_dz = hyn_z_1*(hyn_z1_1 + hyn_z2_1 + hyn_z3_1);

%--------%--------%--------%--------%--------%--------%--------%----------
% Line along x - axis
%-%--------%--------%--------%--------%a--------%--------%--------%--------
xp1_1 = -0.8e-3 - 5*k;
xp2_1 = 0.8e-3 + 5*k;
xn1_1 = -1e-3 - 5*k;
xn2_1 = 1e-3 + 5*k;
a_yp_1 = 2.675e-3;          %Distance of coil from (0,0)
a_yn_1 = -2.675e-3;

k_xp_1 = 1/(4*pi*((a_yp_1-y)^2+z^2));
k_1xp_1 = (xp2_1-x)/((xp2_1-x)^2+(a_yp_1-y)^2+z^2)^0.5;
k_2xp_1 = (xp1_1-x)/((xp1_1-x)^2+(a_yp_1-y)^2+z^2)^0.5;

k_xn_1 = 1/(4*pi*((a_yn_1-y)^2+z^2));
k_1xn_1 = (xn2_1-x)/((xn2_1-x)^2+(a_yn_1-y)^2+z^2)^0.5;
k_2xn_1 = (xn1_1-x)/((xn1_1-x)^2+(a_yn_1-y)^2+z^2)^0.5;

k_1xp_3 = (xp2_1-x)/((xp2_1-x)^2+(a_yp_1-y)^2+z^2)^1.5;
k_2xp_3 = (xp1_1-x)/((xp1_1-x)^2+(a_yp_1-y)^2+z^2)^1.5;

k_1xn_3 = (xn2_1-x)/((xn2_1-x)^2+(a_yn_1-y)^2+z^2)^1.5;
k_2xn_3 = (xn1_1-x)/((xn1_1-x)^2+(a_yn_1-y)^2+z^2)^1.5;

hxp_x_1 = -(z*k_xp_1*(a_yp_1-y))*I*m0;
hxp_x1_1 = (k_xp_1*(k_1xp_1 - k_2xp_1))*2*4*pi;
hxp_x2_1 = k_1xp_3 - k_2xp_3;
dByp_1_dy = hxp_x_1*(hxp_x1_1 + hxp_x2_1);

hxp_z_1 = (k_xp_1)*I*m0;
hxp_z1_1 = (k_1xp_1 - k_2xp_1)*(-1);
hxp_z2_1 = (k_xp_1*(k_1xp_1 - k_2xp_1)*(z^2))*4*pi*2;
hxp_z3_1 = (k_1xp_3 - k_2xp_3)*(z^2);
dByp_1_dz = hxp_z_1*(hxp_z1_1 + hxp_z2_1 + hxp_z3_1);

hxn_x_1 = -(z*k_xn_1*(a_yn_1-y))*I*m0*(-1);
hxn_x1_1 = (k_xn_1*(k_1xn_1 - k_2xn_1))*2*4*pi;
hxn_x2_1 = k_1xn_3 - k_2xn_3;
dByn_1_dy = hxn_x_1*(hxn_x1_1 + hxn_x2_1);

hxn_z_1 = (k_xn_1)*I*m0*(-1);
hxn_z1_1 = (k_1xn_1 - k_2xn_1)*(-1);
hxn_z2_1 = (k_xn_1*(k_1xn_1 - k_2xn_1)*(z^2))*4*pi*2;
hxn_z3_1 = (k_1xn_3 - k_2xn_3)*(z^2);
dByn_1_dz = hxn_z_1*(hxn_z1_1 + hxn_z2_1 + hxn_z3_1);

F_xx_6 = vol_cy * Magentization* (dBxp_1_dx + dBxn_1_dx)/m0;
F_xz_6 = vol_cy * Magentization* (dBxp_1_dz + dBxn_1_dz)/m0;
F_yy_6 = vol_cy * Magentization* (dByp_1_dy + dByn_1_dy)/m0;
F_yz_6 = vol_cy * Magentization* (dByp_1_dz + dByn_1_dz)/m0;
end
